simulink model "NDI"  (R2022a)
settings: Solver=ode4  StartTime=0  StopTime=100  FixedStep=fcs.Ts  RelTol=1e-3
undefined symbols (not defined in the file or in its folder): Aactuator, ac, AeroCoeff, ControlAllocation, DUmax, DUmin, EngineTable, F, fcs, ft, g, hground, IC, kg, LandingGear, Light, m, MIL, Mode_deflection_aileron, Mode_deflection_elevator, Mode_deflection_rudder, Mode_deflection_TVC_y, Mode_deflection_TVC_z, N, Ninv_2nozzle, Ninv_no_nozzle, PIController, s, Sensor, sigbuilder_block, slug, state0, sysID_DAQ, sysID_OBES, Umax_2nozzle, Umax_no_nozzle, Umin_2nozzle, Umin_no_nozzle, WMM2020
libraries: aerolibconvert2 x31, slpidlib x11, simulink x6, sharedutil x4, aerolibatmos2 x3, aerolibwind2 x3, aerolibbdyn x3, aerolibgravity2 x2, sharedtransform x1
(part 5 of 13)

== system NDI/F-16 Vehicle Systems Model/pqr NDI Controller ==
  note: $\hat{L}, \hat{M}, \hat{N}$
  note: 【有向量噴嘴控制】
      | (註：有/無向量噴嘴的差異之處在於 "粉紅色模塊" 的內容)
  note: 1  gp_dra1
      |     gp_dla1
      |     gp_dre1
      |     gp_dle1
      |     gp_dr1
      |     gp_dra2
      |     gp_dla2
      |     gp_dre2
      |     gp_dle2
      |     gp_dr2
      |
      | 11 gq_dra
      |      gq_dla
      |      gq_dre
      |      gq_dle
      |
      | 15 gr_dra1
      |      gr_dla1
      |      gr_dre1
      |      gr_dle1
      |      gr_dr1
      |      gr_dra2
      |      gr_dla2
      |      gr_dre2
      |      gr_dle2
      |      gr_dr2
  note: $g_1 {\left({\overset{-}{x} }_1 \right)}={\left[\begin{array}{ccccccccc} g_{p_{\delta_{ra} } } & g_{p_{\delta_{la} } } & g_{p_{\delta_{re} } } & g_{p_{\delta_{le} } } & g_{p_{\delta_r } } & g_{p_{\delta_{ry} } } & g_{p_{\delta_{rz} } } & g_{p_{\delta_{ly} } } & g_{p_{\delta_{lz} } } \\ g_{q_{\delta_{ra} } } & g_{q_{\delta_{la} } } & g_{q_{\delta_{re} } } & g_{q_{\delta_{le} } } & 0 & g_{q_{\delta_{ry} } } & 0 & g_{q_{\delta_{ly} } } & 0 \\ g_{r_{\delta_{ra} } } & g_{r_{\delta_{la} } } & g_{r_{\delta_{re} } } & g_{r_{\delta_{le} } } & g_{r_{\delta_r } } & g_{r_{\delta_{ry} } } & g_{r_{\delta_{rz} } } & g_{r_{\delta_{ly} } } & g_{r_{\delta_{lz} } } \end{array}\right]}$
  note: 選擇偏轉模式
  coef M : Inport
  control g : Inport  Port=2
  pqr dot desire : Inport  Port=3
  p q r : Inport  Port=4
  In Bus Element : Inport  Port=5  PortName=PlantData  Element=PropBus.T
  In Bus Element12 : Inport  Port=5  PortName=PlantData  Element=alpha
  In Bus Element3 : Inport  Port=5  PortName=PlantData  Element=Vt
  In Bus Element14 : Inport  Port=5  PortName=PlantData  Element=altitude
  " f1" : MATLAB Function  TreatAsAtomicUnit=on
  Angle Conversion : aerolibconvert2/Angle Conversion  IU=rad  OU=deg
  Constant : Constant  Value=0
  Constant1 : Constant  Value=N
  Control Allocation : Subsystem
  Demux : Demux  Outputs=9
  Ix(slug*ft^2)1 : Constant  Value=ac.Ix
  Ixz(slug*ft^2)1 : Constant  Value=ac.Ixz
  Iy(slug*ft^2)1 : Constant  Value=ac.Iy
  Iz(slug*ft^2)1 : Constant  Value=ac.Iz
  MakeINMAT : Subsystem
  Mode_deflection : Subsystem
  Sum : Sum  Inputs=+-|
  To Workspace3 : ToWorkspace  VariableName=upast  SaveFormat=Timeseries  SampleTime=-1
  Unit Delay : UnitDelay  InitialCondition=[0 0 0 0 0 0 0 0 0]  SampleTime=fcs.Ts  HasFrameUpgradeWarning=on
  control matrix g1 : Subsystem
  left_rudder : Terminator
  "TVC_ry " : Outport  VectorParamsAs1DForOutWhenUnconnected=off
  TVC_rz : Outport  Port=2  VectorParamsAs1DForOutWhenUnconnected=off
  "TVC_ly " : Outport  Port=3  VectorParamsAs1DForOutWhenUnconnected=off
  "TVC_lz " : Outport  Port=4  VectorParamsAs1DForOutWhenUnconnected=off
  right_aileron : Outport  Port=5  VectorParamsAs1DForOutWhenUnconnected=off
  left_aileron : Outport  Port=6  VectorParamsAs1DForOutWhenUnconnected=off
  right_elevator : Outport  Port=7  VectorParamsAs1DForOutWhenUnconnected=off
  left_elevator : Outport  Port=8  VectorParamsAs1DForOutWhenUnconnected=off
  rudder : Outport  Port=9  VectorParamsAs1DForOutWhenUnconnected=off
  wires:
  coef M/1 -> " f1"/1(moments)
  p q r/1 -> " f1"/2(pqr)
  " f1"/1(f1) -> Sum/2
  pqr dot desire/1 -> Sum/1
  In Bus Element/1 -> control matrix g1/2(Thrust T)
  control g/1 -> control matrix g1/1(coef g)
  Iy(slug*ft^2)1/1 -> " f1"/4(Iy)
  Ix(slug*ft^2)1/1 -> " f1"/3(Ix)
  Iz(slug*ft^2)1/1 -> " f1"/5(Iz)
  Ixz(slug*ft^2)1/1 -> " f1"/6(Ixz)
  MakeINMAT/1(IN_MAT) -> Control Allocation/1(IN_MAT1)
  Sum/1 -> Control Allocation/5(y_bar), MakeINMAT/1(f1)
  control matrix g1/1(g1) -> Control Allocation/6(g1), MakeINMAT/2(g1)
  Control Allocation/1(Du) -> Unit Delay/1, To Workspace3/1, Demux/1
  Unit Delay/1 -> MakeINMAT/3(In3)
  In Bus Element3/1 -> Control Allocation/3(Vt (ft/s))
  In Bus Element14/1 -> Control Allocation/4(altitude (ft))
  Constant/1 -> Mode_deflection/6(dlr)
  Constant1/1 -> Control Allocation/7(N)
  Demux/9 -> Mode_deflection/10(dlz)
  Demux/1 -> Mode_deflection/1(dra)
  Demux/2 -> Mode_deflection/2(dla)
  Demux/5 -> Mode_deflection/5(drr)
  Demux/4 -> Mode_deflection/4(dle)
  Demux/8 -> Mode_deflection/9(dly)
  Demux/6 -> Mode_deflection/7(dry)
  Demux/3 -> Mode_deflection/3(dre)
  Demux/7 -> Mode_deflection/8(drz)
  Mode_deflection/9("TVC_ly ") -> "TVC_ly "/1
  Mode_deflection/10("TVC_lz ") -> "TVC_lz "/1
  Mode_deflection/7("TVC_ry ") -> "TVC_ry "/1
  Mode_deflection/8(TVC_rz) -> TVC_rz/1
  Mode_deflection/2(left_aileron) -> left_aileron/1
  Mode_deflection/4(left_elevator) -> left_elevator/1
  Mode_deflection/6(left_rudder) -> left_rudder/1
  Mode_deflection/1(right_aileron) -> right_aileron/1
  Mode_deflection/3(right_elevator) -> right_elevator/1
  Mode_deflection/5(rudder) -> rudder/1
  In Bus Element12/1 -> Angle Conversion/1
  Angle Conversion/1 -> Control Allocation/2(alpha (deg))

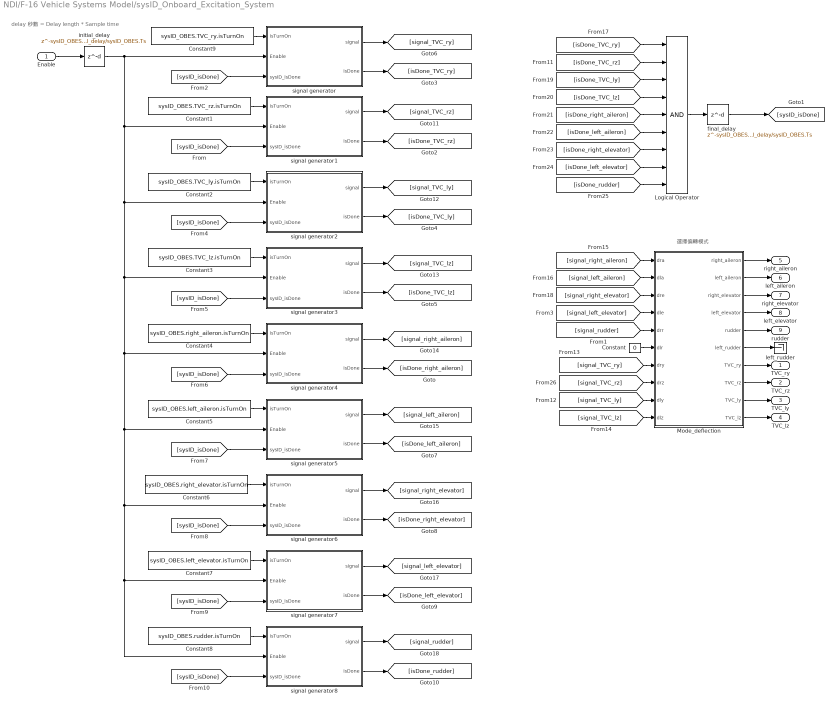
== system NDI/F-16 Vehicle Systems Model/sysID_Onboard_Excitation_System ==
  note: delay 秒數 = Delay length * Sample time
  note: 選擇偏轉模式
  Enable : Inport
  Constant : Constant  Value=0
  Constant1 : Constant  Value=sysID_OBES.TVC_rz.isTurnOn
  Constant2 : Constant  Value=sysID_OBES.TVC_ly.isTurnOn
  Constant3 : Constant  Value=sysID_OBES.TVC_lz.isTurnOn
  Constant4 : Constant  Value=sysID_OBES.right_aileron.isTurnOn
  Constant5 : Constant  Value=sysID_OBES.left_aileron.isTurnOn
  Constant6 : Constant  Value=sysID_OBES.right_elevator.isTurnOn
  Constant7 : Constant  Value=sysID_OBES.left_elevator.isTurnOn
  Constant8 : Constant  Value=sysID_OBES.rudder.isTurnOn
  Constant9 : Constant  Value=sysID_OBES.TVC_ry.isTurnOn
  Logical Operator : Logic  Inputs=9  AllPortsSameDT=off  OutDataTypeStr=boolean
  Mode_deflection : Subsystem
  final_delay : Delay  DelayLength=sysID_OBES.final_delay/sysID_OBES.Ts  SampleTime=sysID_OBES.Ts
  initial_delay : Delay  DelayLength=sysID_OBES.initial_delay/sysID_OBES.Ts  SampleTime=sysID_OBES.Ts
  left_rudder : Terminator
  signal generator : Subsystem  TreatAsAtomicUnit=on
  signal generator1 : Subsystem  TreatAsAtomicUnit=on
  signal generator2 : Subsystem  TreatAsAtomicUnit=on
  signal generator3 : Subsystem  TreatAsAtomicUnit=on
  signal generator4 : Subsystem  TreatAsAtomicUnit=on
  signal generator5 : Subsystem  TreatAsAtomicUnit=on
  signal generator6 : Subsystem  TreatAsAtomicUnit=on
  signal generator7 : Subsystem  TreatAsAtomicUnit=on
  signal generator8 : Subsystem  TreatAsAtomicUnit=on
  TVC_ry : Outport
  TVC_rz : Outport  Port=2
  TVC_ly : Outport  Port=3
  TVC_lz : Outport  Port=4
  right_aileron : Outport  Port=5
  left_aileron : Outport  Port=6
  right_elevator : Outport  Port=7
  left_elevator : Outport  Port=8
  rudder : Outport  Port=9
  wires:
  Logical Operator/1 -> final_delay/1
  final_delay/1 -> [sysID_isDone]
  signal generator1/2(isDone) -> [isDone_TVC_rz]
  [sysID_isDone] -> signal generator1/3(sysID_isDone)
  Enable/1 -> initial_delay/1
  signal generator/2(isDone) -> [isDone_TVC_ry]
  [sysID_isDone] -> signal generator/3(sysID_isDone)
  signal generator2/2(isDone) -> [isDone_TVC_ly]
  [sysID_isDone] -> signal generator2/3(sysID_isDone)
  signal generator3/2(isDone) -> [isDone_TVC_lz]
  [sysID_isDone] -> signal generator3/3(sysID_isDone)
  signal generator4/2(isDone) -> [isDone_right_aileron]
  [sysID_isDone] -> signal generator4/3(sysID_isDone)
  signal generator5/2(isDone) -> [isDone_left_aileron]
  [sysID_isDone] -> signal generator5/3(sysID_isDone)
  [sysID_isDone] -> signal generator6/3(sysID_isDone)
  signal generator6/2(isDone) -> [isDone_right_elevator]
  [sysID_isDone] -> signal generator7/3(sysID_isDone)
  signal generator7/2(isDone) -> [isDone_left_elevator]
  [sysID_isDone] -> signal generator8/3(sysID_isDone)
  initial_delay/1 -> signal generator1/2(Enable), signal generator2/2(Enable), signal generator3/2(Enable), signal generator4/2(Enable), signal generator5/2(Enable), signal generator6/2(Enable), signal generator8/2(Enable), signal generator7/2(Enable), signal generator/2(Enable)
  signal generator8/2(isDone) -> [isDone_rudder]
  Constant1/1 -> signal generator1/1(isTurnOn)
  Constant2/1 -> signal generator2/1(isTurnOn)
  Constant3/1 -> signal generator3/1(isTurnOn)
  Constant4/1 -> signal generator4/1(isTurnOn)
  Constant5/1 -> signal generator5/1(isTurnOn)
  Constant6/1 -> signal generator6/1(isTurnOn)
  Constant7/1 -> signal generator7/1(isTurnOn)
  Constant8/1 -> signal generator8/1(isTurnOn)
  Constant/1 -> Mode_deflection/6(dlr)
  Constant9/1 -> signal generator/1(isTurnOn)
  [isDone_TVC_ly] -> Logical Operator/3
  [isDone_TVC_lz] -> Logical Operator/4
  [isDone_right_aileron] -> Logical Operator/5
  [isDone_left_aileron] -> Logical Operator/6
  [isDone_right_elevator] -> Logical Operator/7
  [isDone_left_elevator] -> Logical Operator/8
  [signal_TVC_ry] -> Mode_deflection/7(dry)
  [isDone_rudder] -> Logical Operator/9
  [signal_TVC_ly] -> Mode_deflection/9(dly)
  [isDone_TVC_ry] -> Logical Operator/1
  [signal_TVC_lz] -> Mode_deflection/10(dlz)
  [signal_right_aileron] -> Mode_deflection/1(dra)
  [signal_left_aileron] -> Mode_deflection/2(dla)
  [signal_right_elevator] -> Mode_deflection/3(dre)
  [signal_left_elevator] -> Mode_deflection/4(dle)
  [signal_rudder] -> Mode_deflection/5(drr)
  [signal_TVC_rz] -> Mode_deflection/8(drz)
  [isDone_TVC_rz] -> Logical Operator/2
  Mode_deflection/9("TVC_ly ") -> TVC_ly/1
  Mode_deflection/10("TVC_lz ") -> TVC_lz/1
  Mode_deflection/7("TVC_ry ") -> TVC_ry/1
  Mode_deflection/8(TVC_rz) -> TVC_rz/1
  Mode_deflection/2(left_aileron) -> left_aileron/1
  Mode_deflection/4(left_elevator) -> left_elevator/1
  Mode_deflection/6(left_rudder) -> left_rudder/1
  Mode_deflection/1(right_aileron) -> right_aileron/1
  Mode_deflection/3(right_elevator) -> right_elevator/1
  Mode_deflection/5(rudder) -> rudder/1
  signal generator1/1(signal) -> [signal_TVC_rz]
  signal generator2/1(signal) -> [signal_TVC_ly]
  signal generator3/1(signal) -> [signal_TVC_lz]
  signal generator4/1(signal) -> [signal_right_aileron]
  signal generator5/1(signal) -> [signal_left_aileron]
  signal generator6/1(signal) -> [signal_right_elevator]
  signal generator7/1(signal) -> [signal_left_elevator]
  signal generator8/1(signal) -> [signal_rudder]
  signal generator/1(signal) -> [signal_TVC_ry]

== system NDI/F-16 Vehicle Systems Model/μαβ NDI Controller ==
  aero F : Inport
  μαβ dot desire : Inport  Port=2
  LGxyz : Inport  Port=3
  gravity : Inport  Port=4
  In Bus Element2 : Inport  Port=5  PortName=AirData  Element=alpha
  In Bus Element4 : Inport  Port=5  PortName=AirData  Element=alpha
  In Bus Element3 : Inport  Port=5  PortName=AirData  Element=beta
  In Bus Element5 : Inport  Port=5  PortName=AirData  Element=beta
  In Bus Element6 : Inport  Port=5  PortName=AirData  Element=mu
  In Bus Element7 : Inport  Port=5  PortName=AirData  Element=Vt
  In Bus Element8 : Inport  Port=5  PortName=AirData  Element=gamma
  In Bus Element : Inport  Port=6  PortName=PlantData  Element=PropBus.T
  In Bus Element1 : Inport  Port=6  PortName=PlantData  Element=chi
  Mux : Mux  Inputs=5
  Sum : Sum  Inputs=+-|
  attitude NDI : MATLAB Function  TreatAsAtomicUnit=on
  command matrix : Subsystem
  f2 : Subsystem
  pc : Outport  VectorParamsAs1DForOutWhenUnconnected=off
  qc : Outport  Port=2  VectorParamsAs1DForOutWhenUnconnected=off
  rc : Outport  Port=3  VectorParamsAs1DForOutWhenUnconnected=off
  D : Outport  Port=4  VectorParamsAs1DForOutWhenUnconnected=off
  Y : Outport  Port=5  VectorParamsAs1DForOutWhenUnconnected=off
  L : Outport  Port=6  VectorParamsAs1DForOutWhenUnconnected=off
  wires:
  f2/1(f2) -> Sum/2
  μαβ dot desire/1 -> Sum/1
  Sum/1 -> attitude NDI/1(y_bar)
  attitude NDI/1(p_c) -> pc/1
  attitude NDI/2(q_c) -> qc/1
  attitude NDI/3(r_c) -> rc/1
  command matrix/1(g2) -> attitude NDI/2(g2)
  Mux/1 -> f2/1(aero V)  "V, α, β, μ, γ"
  In Bus Element/1 -> f2/4(Thrust)
  aero F/1 -> f2/2(X,Y,Z)
  f2/2(D) -> D/1
  f2/3(Y) -> Y/1
  f2/4(L) -> L/1
  gravity/1 -> f2/3(gravity)
  In Bus Element2/1 -> command matrix/1(α)
  In Bus Element3/1 -> command matrix/2(β)
  In Bus Element5/1 -> Mux/3
  In Bus Element4/1 -> Mux/2
  In Bus Element6/1 -> Mux/4
  In Bus Element7/1 -> Mux/1
  In Bus Element8/1 -> Mux/5
  LGxyz/1 -> f2/5(LGxyz)
  In Bus Element1/1 -> f2/6(chi)

== system NDI/F-16 Vehicle Systems Model/庭宇 6.3節短場降落(模擬秒數設定:inf) ==
  Demux : Demux  Tag=STV Demux  Outputs=5
      settings: DisplayOption=none
  FromWs : FromWorkspace  Tag=STV FromWs  VariableName=tuvar
      SigBuilderData=|
      | common.afterFinalStr = 'Extrapolate'
      | common.sampleTime = 0
      | dataSet.timeRange = [0 120]
      | dataSet.name = 'Group 1'
      | sbobj.Groups.Name = 'Group 1'
      | sbobj.Groups.Signals(1).Name = 'Vt'
      | sbobj.Groups.Signals(1).XData = [0 5 6.2 7.35 8.3 9.05 10.05 11.2 13.1 14.75 15 16.85 18.75 19.63 20 22.2 23.5 25 26.65 30 31.65 40 50 60 67.4 80 94.8 107.7 120]
      | sbobj.Groups.Signals(1).YData = [287 287 286.6 286 285 284.6 283.9 283.4 281.8 279.8 279.4 277 274.8 273.8 273.3 270.3 269 268 266.5 264 263 258 252 248 246 220 197 110 0]
      | sbobj.Groups.Signals(2).Name = 'y_ft'
      | sbobj.Groups.Signals(2).XData = [0 120]
      | sbobj.Groups.Signals(2).YData = [0 0]
      | sbobj.Groups.Signals(3).Name = 'h_ft'
      | sbobj.Groups.Signals(3).XData = [0 60 80.12 94 100 120]
      | sbobj.Groups.Signals(3).YData = [1000 100 6.1418 6.1418 5.9161 5.9161]
      | sbobj.Groups.Signals(4).Name = 'SB_deg'
      | sbobj.Groups.Signals(4).XData = [0 100 100 120]
      | sbobj.Groups.Signals(4).YData = [40 40 60 60]
      | sbobj.Groups.Signals(5).Name = 'LandingGear_down'
      | sbobj.Groups.Signals(5).XData = [0 120]
      | sbobj.Groups.Signals(5).YData = [1 1]
      | sbobj.Groups.TimeRange = [0 120]
  Vt : Outport  Tag=STV Outport  VectorParamsAs1DForOutWhenUnconnected=off
  y_ft : Outport  Tag=STV Outport  Port=2  VectorParamsAs1DForOutWhenUnconnected=off
  h_ft : Outport  Tag=STV Outport  Port=3  VectorParamsAs1DForOutWhenUnconnected=off
  SB_deg : Outport  Tag=STV Outport  Port=4
  LandingGear_down : Outport  Tag=STV Outport  Port=5
  wires:
  FromWs/1 -> Demux/1
  Demux/1 -> Vt/1
  Demux/2 -> y_ft/1
  Demux/3 -> h_ft/1
  Demux/4 -> SB_deg/1
  Demux/5 -> LandingGear_down/1

== system NDI/F-16 Vehicle Systems Model/落葉飄完整版(碩論6.7)1 ==
  Demux : Demux  Tag=STV Demux  Outputs=6
      settings: DisplayOption=none
  FromWs : FromWorkspace  Tag=STV FromWs  VariableName=tuvar
      SigBuilderData=|
      | common.afterFinalStr = 'Extrapolate'
      | common.sampleTime = 0
      | dataSet.timeRange = [0 70]
      | dataSet.name = 'Group 5'
      | sbobj.Groups.Name = 'Group 5'
      | sbobj.Groups.Signals(1).Name = 'thrust'
      | sbobj.Groups.Signals(1).XData = [0 2 4 5 6 8 9 10 12 20 25 30 35 40 70]
      | sbobj.Groups.Signals(1).YData = [5100 5100 600 200 200 200 265 3500 3500 3500 6000 15200 15200 10000 10000]
      | sbobj.Groups.Signals(2).Name = 'mu'
      | sbobj.Groups.Signals(2).XData = [0 2 8 10 12 20 30 40 55 67 70]
      | sbobj.Groups.Signals(2).YData = [0 0 0 0 0 90 90 0 80 0 0]
      | sbobj.Groups.Signals(3).Name = 'alpha'
      | sbobj.Groups.Signals(3).XData = [0 1 2 3 10 35 37 60 70]
      | sbobj.Groups.Signals(3).YData = [7 30 31 60 70 70 10 20 20]
      | sbobj.Groups.Signals(4).Name = 'beta'
      | sbobj.Groups.Signals(4).XData = [0 8 70]
      | sbobj.Groups.Signals(4).YData = [0 0 0]
      | sbobj.Groups.Signals(5).Name = 'speed brake'
      | sbobj.Groups.Signals(5).XData = [0 70]
      | sbobj.Groups.Signals(5).YData = [0 0]
      | sbobj.Groups.Signals(6).Name = 'LandingGear_down'
      | sbobj.Groups.Signals(6).XData = [0 70]
      | sbobj.Groups.Signals(6).YData = [1 1]
      | sbobj.Groups.TimeRange = [0 70]
  thrust : Outport  Tag=STV Outport
  mu : Outport  Tag=STV Outport  Port=2  VectorParamsAs1DForOutWhenUnconnected=off
  alpha : Outport  Tag=STV Outport  Port=3  VectorParamsAs1DForOutWhenUnconnected=off
  beta : Outport  Tag=STV Outport  Port=4  VectorParamsAs1DForOutWhenUnconnected=off
  speed brake : Outport  Tag=STV Outport  Port=5
  LandingGear_down : Outport  Tag=STV Outport  Port=6
  wires:
  FromWs/1 -> Demux/1
  Demux/1 -> thrust/1
  Demux/2 -> mu/1
  Demux/3 -> alpha/1
  Demux/4 -> beta/1
  Demux/5 -> speed brake/1
  Demux/6 -> LandingGear_down/1

== system NDI/F-16 Vehicle Systems Model/Aerodynamic1/Creating    qbar // ps ==
  h (ft) : Inport
  Vt (ft/s) : Inport  Port=2
  Constant2 : Constant
  Constant3 : Constant  Value=390
  Constant6 : Constant  Value=4.14
  Math Function : Math  Operator=pow  SignedPower=on
  Math Function1 : Math  Operator=square  SignedPower=on
  Product : Product  Inputs=/*  InputSameDT=on  SaturateOnIntegerOverflow=on  OutDataTypeStr=Inherit: Same as first input
  Product5 : Product  Inputs=**  InputSameDT=on  SaturateOnIntegerOverflow=on  OutDataTypeStr=Inherit: Same as first input
  Product6 : Product  Inputs=**  InputSameDT=on  SaturateOnIntegerOverflow=on  OutDataTypeStr=Inherit: Same as first input
  Sum3 : Sum  Inputs=+-|  InputSameDT=on  SaturateOnIntegerOverflow=on  OutDataTypeStr=Inherit: Same as first input
  Switch : Switch  Threshold=35000
  r2d2 : Gain  Gain=0.703e-5  SaturateOnIntegerOverflow=on  OutDataTypeStr=Inherit: Same as input  ParamDataTypeStr=Inherit: Same as input
  r2d3 : Gain  Gain=519  SaturateOnIntegerOverflow=on  OutDataTypeStr=Inherit: Same as input  ParamDataTypeStr=Inherit: Same as input
  r2d4 : Gain  Gain=0.5  SaturateOnIntegerOverflow=on  OutDataTypeStr=Inherit: Same as input  ParamDataTypeStr=Inherit: Same as input
  r2d5 : Gain  Gain=1715  SaturateOnIntegerOverflow=on  OutDataTypeStr=Inherit: Same as input  ParamDataTypeStr=Inherit: Same as input
  rho0 : Gain  Gain=2.377e-3  SaturateOnIntegerOverflow=on  OutDataTypeStr=Inherit: Same as input  ParamDataTypeStr=Inherit: Same as input
  qbar / ps : Outport  VectorParamsAs1DForOutWhenUnconnected=off
  wires:
  h (ft)/1 -> r2d2/1, Switch/2
  Sum3/1 -> Math Function/1, r2d3/1  "tfac"
  Constant3/1 -> Switch/1
  r2d3/1 -> Switch/3
  Constant6/1 -> Math Function/2
  rho0/1 -> Product5/1, Product6/2  "rho"
  r2d2/1 -> Sum3/2
  Constant2/1 -> Sum3/1
  Math Function/1 -> rho0/1
  Math Function1/1 -> Product5/2
  Switch/1 -> r2d5/1  "temp"
  r2d5/1 -> Product6/1
  Product6/1 -> Product/1  "ps"
  Product5/1 -> r2d4/1  "qbar"
  Product/1 -> qbar / ps/1
  Vt (ft/s)/1 -> Math Function1/1  "Vt (ft/s)"
  r2d4/1 -> Product/2

== system NDI/F-16 Vehicle Systems Model/Aerodynamic1/ISP  ==
  note: 1 T
      | 2 a (Speed of sound)
      | 3 P
      | 4 rho
      | 5 g
      | 6 mu (Coefficient of viscosity)
  h (ft) : Inport
  Vt (ft/s) : Inport  Port=2
  Demux : Demux  Outputs=[1,1,1,1,1,1]
      settings: DisplayOption=none
  Divide1 : Product  Inputs=*/
  Length Conversion : aerolibconvert2/Length Conversion  IU=ft  OU=m
  MATLAB Function : MATLAB Function  TreatAsAtomicUnit=on
  Product : Product
  Square : Math  Operator=square  SignedPower=on
  r2d1 : Gain  Gain=0.5  SaturateOnIntegerOverflow=on  OutDataTypeStr=Inherit: Same as input  ParamDataTypeStr=Inherit: Same as input
  r2d3 : Gain  Gain=3.2808399  SaturateOnIntegerOverflow=on  OutDataTypeStr=Inherit: Same as input  ParamDataTypeStr=Inherit: Same as input
  r2d4 : Gain  Gain=0.00194032033  SaturateOnIntegerOverflow=on  OutDataTypeStr=Inherit: Same as input  ParamDataTypeStr=Inherit: Same as input
  T(K) : Outport  VectorParamsAs1DForOutWhenUnconnected=off
  "Mach " : Outport  Port=2  VectorParamsAs1DForOutWhenUnconnected=off
  P(HPa) : Outport  Port=3  VectorParamsAs1DForOutWhenUnconnected=off
  "qbar " : Outport  Port=4  VectorParamsAs1DForOutWhenUnconnected=off
  rho : Outport  Port=5  VectorParamsAs1DForOutWhenUnconnected=off
  g (m/s^2) : Outport  Port=6  VectorParamsAs1DForOutWhenUnconnected=off
  mu : Outport  Port=7  VectorParamsAs1DForOutWhenUnconnected=off
  wires:
  r2d3/1 -> Divide1/2
  r2d1/1 -> Product/2
  Demux/4 -> rho/1, r2d4/1  "rho(kg/m^3)"
  Demux/2 -> r2d3/1  "a(m/s)"
  Demux/1 -> T(K)/1  "T(K)"
  r2d4/1 -> r2d1/1
  Divide1/1 -> "Mach "/1
  Demux/5 -> g (m/s^2)/1  "g (m/s^2)"
  Demux/6 -> mu/1  "mu"
  Product/1 -> "qbar "/1
  Square/1 -> Product/1
  Vt (ft/s)/1 -> Square/1, Divide1/1
  Demux/3 -> P(HPa)/1  "P(Pa)"
  h (ft)/1 -> Length Conversion/1
  Length Conversion/1 -> MATLAB Function/1(h)
  MATLAB Function/1(ISP_output) -> Demux/1

== system NDI/F-16 Vehicle Systems Model/Aerodynamic1/NDI Aerofynamic Coefficients ==
  note: leading-edge flaps
      | 前緣襟翼
  note: speed brake
      | 減速板
  note: Total Velocity
  note: 未建模，缺少數據
  note: ${\left(1-\frac{\delta_{LEF} }{25°}\right)}$
  alpha (deg) : Inport
  beta (deg) : Inport  Port=2
  LEF (deg) : Inport  Port=3
  right elevator (deg) : Inport  Port=4
  left elevator (deg) : Inport  Port=5
  right alieron (deg) : Inport  Port=6
  left alieron (deg) : Inport  Port=7
  rudder (deg) : Inport  Port=8
  SB (deg) : Inport  Port=9  Unit=deg
  Vt (ft/s) : Inport  Port=10
  p (rad/s) : Inport  Port=11
  q (rad/s) : Inport  Port=12
  r (rad/s) : Inport  Port=13
  GearAngle : Inport  Port=14
  h_AGL : Inport  Port=15
  Add : Sum  Inputs=-+
  CXT : Subsystem
  CYT : Subsystem
  CZT : Subsystem
  ClT : Subsystem
  CmT : Subsystem
  CnT : Subsystem
  Constant3 : Constant
  Divide2 : Product  Inputs=**/
  Divide3 : Product  Inputs=**/
  Divide4 : Product  Inputs=**/
  Gain1 : Gain  Gain=2
  Ground Effects : Subsystem  Commented=on
  Landing Gear Effects : Subsystem  Commented=on
  Mux : Mux  Inputs=2
  Mux1 : Mux  Inputs=2
  Terminator : Terminator  Commented=on
  Terminator1 : Terminator  Commented=on
  b(ft) : Constant  Value=ac.b
  cbar(ft) : Constant  Value=ac.cbar
  center of gravity as a fraction of cbar : Constant  Value=ac.x_cg
  r2d1 : Gain  Gain=1/25  SaturateOnIntegerOverflow=on  OutDataTypeStr=Inherit: Same as input  ParamDataTypeStr=Inherit: Same as input
  r2d2 : Gain  Gain=1/60  SaturateOnIntegerOverflow=on  OutDataTypeStr=Inherit: Same as input  ParamDataTypeStr=Inherit: Same as input
  r2d3 : Gain  Gain=1/20  SaturateOnIntegerOverflow=on  OutDataTypeStr=Inherit: Same as input  ParamDataTypeStr=Inherit: Same as input
  r2d4 : Gain  Gain=1/30  SaturateOnIntegerOverflow=on  OutDataTypeStr=Inherit: Same as input  ParamDataTypeStr=Inherit: Same as input
  r2d5 : Gain  Gain=1/20  SaturateOnIntegerOverflow=on  OutDataTypeStr=Inherit: Same as input  ParamDataTypeStr=Inherit: Same as input
  reference center of gravity as a fraction of cbar : Constant  Value=ac.x_cg_ref
  CX_T : Outport  VectorParamsAs1DForOutWhenUnconnected=off
  CY_T : Outport  Port=2  VectorParamsAs1DForOutWhenUnconnected=off
  CZ_T : Outport  Port=3  VectorParamsAs1DForOutWhenUnconnected=off
  Cl_T_hat : Outport  Port=4  VectorParamsAs1DForOutWhenUnconnected=off
  Cm_T_hat : Outport  Port=5  VectorParamsAs1DForOutWhenUnconnected=off
  Cn_T_hat : Outport  Port=6  VectorParamsAs1DForOutWhenUnconnected=off
  gp : Outport  Port=7  VectorParamsAs1DForOutWhenUnconnected=off
  gq : Outport  Port=8  VectorParamsAs1DForOutWhenUnconnected=off
  gr : Outport  Port=9  VectorParamsAs1DForOutWhenUnconnected=off
  wires:
  alpha (deg)/1 -> CXT/1(alpha (deg)), CnT/1(alpha (deg)), CmT/1(alpha (deg)), ClT/1(alpha (deg)), CZT/1(alpha (deg)), CYT/1(alpha (deg))
  beta (deg)/1 -> CXT/2(beta (deg)), CnT/2(beta (deg)), CmT/2(beta (deg)), ClT/2(beta (deg)), CZT/2(beta (deg)), CYT/2(beta (deg))
  right elevator (deg)/1 -> CXT/3(right elevator (deg)), CnT/3(right elevator (deg)), CmT/3(right elevator (deg)), ClT/3(right elevator (deg)), CZT/3(right elevator (deg))
  Vt (ft/s)/1 -> Gain1/1
  p (rad/s)/1 -> Divide4/1  "p"
  q (rad/s)/1 -> Divide2/1  "q"
  r (rad/s)/1 -> Divide3/1  "r"
  b(ft)/1 -> Divide4/2, Divide3/2, CnT/11(b)  "b"
  cbar(ft)/1 -> Divide2/2, CnT/10(cbar)  "cbar"
  Add/1 -> CXT/5(dlef), CnT/5(dlef), CmT/5(dlef), ClT/5(dlef), CZT/5(dlef), CYT/3(dlef)  "dlef"
  left alieron (deg)/1 -> r2d3/1
  rudder (deg)/1 -> r2d4/1
  Divide2/1 -> CXT/6(qc_2v), CZT/6(qc_2v), CmT/6(qc_2v)  "qc_2v"
  r2d4/1 -> CYT/6(drud)
  Divide3/1 -> CnT/6(rb_2v), CYT/7(rb_2v), ClT/6(rb_2v)  "rb_2v"
  Divide4/1 -> CnT/7(pb_2v), CYT/8(pb_2v), ClT/7(pb_2v)  "pb_2v"
  reference center of gravity as a fraction of cbar/1 -> CmT/7(x_cg_ref), CnT/8(x_cg_ref)
  center of gravity as a fraction of cbar/1 -> CmT/8(x_cg), CnT/9(x_cg)
  CZT/1(Cz_tot_plus) -> CmT/10(Cz_tot_plus)
  CZT/2(Cz_tot_minus) -> CmT/11(Cz_tot_minus)
  CYT/2(Cy_tot_n_mom) -> CnT/12(Cy_tot_n_mom)
  CYT/3(Cy_tot_n_da) -> CnT/13(Cy_tot_n_da)
  CYT/4(Cy_tot_n_dr) -> CnT/14(Cy_tot_n_dr)
  SB (deg)/1 -> r2d2/1
  CXT/1(Cx_tot) -> CX_T/1
  CYT/1(Cy_tot) -> CY_T/1
  CZT/5(Cz_tot) -> CZ_T/1
  CnT/1(Cn_tot_hat) -> Cn_T_hat/1
  CmT/1(Cm_tot_hat) -> Cm_T_hat/1
  ClT/1(Cl_tot_hat) -> Cl_T_hat/1
  LEF (deg)/1 -> r2d1/1
  r2d2/1 -> CXT/7(sb), CmT/12(sb), CZT/7(sb)
  Gain1/1 -> Divide3/3, Divide2/3, Divide4/3  "2v"
  Landing Gear Effects/1(Coeff) -> Terminator/1
  h_AGL/1 -> Ground Effects/3(h_AGL)
  Ground Effects/1(Coeff) -> Terminator1/1
  GearAngle/1 -> Landing Gear Effects/3(Landing Gear Angle)
  right alieron (deg)/1 -> r2d5/1
  r2d5/1 -> CXT/8(right aileron), CYT/4(right aileron)
  r2d3/1 -> CYT/5(left aileron), CXT/9(left aileron)
  r2d1/1 -> Add/1
  Constant3/1 -> Add/2
  left elevator (deg)/1 -> CXT/4(left elevator (deg)), CnT/4(left elevator (deg)), CmT/4(left elevator (deg)), ClT/4(left elevator (deg)), CZT/4(left elevator (deg))
  Mux1/1 -> gr/1
  CmT/3(gq) -> gq/1
  CnT/3(gr2) -> Mux1/2
  ClT/3(gr1) -> Mux1/1
  CnT/2(gp2) -> Mux/2
  Mux/1 -> gp/1
  ClT/2(gp1) -> Mux/1
  CZT/6(Cz_tot_hat) -> CmT/9(Cz_tot_hat)
  CYT/5(Cy_tot_n_de) -> CnT/15(Cy_tot_n_de)
  CZT/3(Cz_tot_m_de) -> CmT/13(Cz_tot_m_de)
  CZT/4(Cz_tot_m_da) -> CmT/14(Cz_tot_m_da)

== system NDI/F-16 Vehicle Systems Model/Aerodynamic2/Creating    qbar // ps ==
  h (ft) : Inport
  Vt (ft/s) : Inport  Port=2
  Constant2 : Constant
  Constant3 : Constant  Value=390
  Constant6 : Constant  Value=4.14
  Math Function : Math  Operator=pow  SignedPower=on
  Math Function1 : Math  Operator=square  SignedPower=on
  Product : Product  Inputs=/*  InputSameDT=on  SaturateOnIntegerOverflow=on  OutDataTypeStr=Inherit: Same as first input
  Product5 : Product  Inputs=**  InputSameDT=on  SaturateOnIntegerOverflow=on  OutDataTypeStr=Inherit: Same as first input
  Product6 : Product  Inputs=**  InputSameDT=on  SaturateOnIntegerOverflow=on  OutDataTypeStr=Inherit: Same as first input
  Sum3 : Sum  Inputs=+-|  InputSameDT=on  SaturateOnIntegerOverflow=on  OutDataTypeStr=Inherit: Same as first input
  Switch : Switch  Threshold=35000
  r2d2 : Gain  Gain=0.703e-5  SaturateOnIntegerOverflow=on  OutDataTypeStr=Inherit: Same as input  ParamDataTypeStr=Inherit: Same as input
  r2d3 : Gain  Gain=519  SaturateOnIntegerOverflow=on  OutDataTypeStr=Inherit: Same as input  ParamDataTypeStr=Inherit: Same as input
  r2d4 : Gain  Gain=0.5  SaturateOnIntegerOverflow=on  OutDataTypeStr=Inherit: Same as input  ParamDataTypeStr=Inherit: Same as input
  r2d5 : Gain  Gain=1715  SaturateOnIntegerOverflow=on  OutDataTypeStr=Inherit: Same as input  ParamDataTypeStr=Inherit: Same as input
  rho0 : Gain  Gain=2.377e-3  SaturateOnIntegerOverflow=on  OutDataTypeStr=Inherit: Same as input  ParamDataTypeStr=Inherit: Same as input
  qbar / ps : Outport  VectorParamsAs1DForOutWhenUnconnected=off
  wires:
  h (ft)/1 -> r2d2/1, Switch/2
  Sum3/1 -> Math Function/1, r2d3/1  "tfac"
  Constant3/1 -> Switch/1
  r2d3/1 -> Switch/3
  Constant6/1 -> Math Function/2
  rho0/1 -> Product5/1, Product6/2  "rho"
  r2d2/1 -> Sum3/2
  Constant2/1 -> Sum3/1
  Math Function/1 -> rho0/1
  Math Function1/1 -> Product5/2
  Switch/1 -> r2d5/1  "temp"
  r2d5/1 -> Product6/1
  Product6/1 -> Product/1  "ps"
  Product5/1 -> r2d4/1  "qbar"
  Product/1 -> qbar / ps/1
  Vt (ft/s)/1 -> Math Function1/1  "Vt (ft/s)"
  r2d4/1 -> Product/2

== system NDI/F-16 Vehicle Systems Model/Aerodynamic2/ISP  ==
  note: 1 T
      | 2 a (Speed of sound)
      | 3 P
      | 4 rho
      | 5 g
      | 6 mu (Coefficient of viscosity)
  h (ft) : Inport
  Vt (ft/s) : Inport  Port=2
  Demux : Demux  Outputs=[1,1,1,1,1,1]
      settings: DisplayOption=none
  Divide1 : Product  Inputs=*/
  Length Conversion : aerolibconvert2/Length Conversion  IU=ft  OU=m
  MATLAB Function : MATLAB Function  TreatAsAtomicUnit=on
  Product : Product
  Square : Math  Operator=square  SignedPower=on
  r2d1 : Gain  Gain=0.5  SaturateOnIntegerOverflow=on  OutDataTypeStr=Inherit: Same as input  ParamDataTypeStr=Inherit: Same as input
  r2d3 : Gain  Gain=3.2808399  SaturateOnIntegerOverflow=on  OutDataTypeStr=Inherit: Same as input  ParamDataTypeStr=Inherit: Same as input
  r2d4 : Gain  Gain=0.00194032033  SaturateOnIntegerOverflow=on  OutDataTypeStr=Inherit: Same as input  ParamDataTypeStr=Inherit: Same as input
  T(K) : Outport  VectorParamsAs1DForOutWhenUnconnected=off
  "Mach " : Outport  Port=2  VectorParamsAs1DForOutWhenUnconnected=off
  P(HPa) : Outport  Port=3  VectorParamsAs1DForOutWhenUnconnected=off
  "qbar " : Outport  Port=4  VectorParamsAs1DForOutWhenUnconnected=off
  rho : Outport  Port=5  VectorParamsAs1DForOutWhenUnconnected=off
  g (m/s^2) : Outport  Port=6  VectorParamsAs1DForOutWhenUnconnected=off
  mu : Outport  Port=7  VectorParamsAs1DForOutWhenUnconnected=off
  wires:
  r2d3/1 -> Divide1/2
  r2d1/1 -> Product/2
  Demux/4 -> rho/1, r2d4/1  "rho(kg/m^3)"
  Demux/2 -> r2d3/1  "a(m/s)"
  Demux/1 -> T(K)/1  "T(K)"
  r2d4/1 -> r2d1/1
  Divide1/1 -> "Mach "/1
  Demux/5 -> g (m/s^2)/1  "g (m/s^2)"
  Demux/6 -> mu/1  "mu"
  Product/1 -> "qbar "/1
  Square/1 -> Product/1
  Vt (ft/s)/1 -> Square/1, Divide1/1
  Demux/3 -> P(HPa)/1  "P(Pa)"
  h (ft)/1 -> Length Conversion/1
  Length Conversion/1 -> MATLAB Function/1(h)
  MATLAB Function/1(ISP_output) -> Demux/1

== system NDI/F-16 Vehicle Systems Model/Aerodynamic2/NDI Aerofynamic Coefficients ==
  note: leading-edge flaps
      | 前緣襟翼
  note: speed brake
      | 減速板
  note: Total Velocity
  note: 未建模，缺少數據
  note: ${\left(1-\frac{\delta_{LEF} }{25°}\right)}$
  alpha (deg) : Inport
  beta (deg) : Inport  Port=2
  LEF (deg) : Inport  Port=3
  right elevator (deg) : Inport  Port=4
  left elevator (deg) : Inport  Port=5
  right alieron (deg) : Inport  Port=6
  left alieron (deg) : Inport  Port=7
  rudder (deg) : Inport  Port=8
  SB (deg) : Inport  Port=9  Unit=deg
  Vt (ft/s) : Inport  Port=10
  p (rad/s) : Inport  Port=11
  q (rad/s) : Inport  Port=12
  r (rad/s) : Inport  Port=13
  GearAngle : Inport  Port=14
  h_AGL : Inport  Port=15
  Add : Sum  Inputs=-+
  CXT : Subsystem
  CYT : Subsystem
  CZT : Subsystem
  ClT : Subsystem
  CmT : Subsystem
  CnT : Subsystem
  Constant3 : Constant
  Divide2 : Product  Inputs=**/
  Divide3 : Product  Inputs=**/
  Divide4 : Product  Inputs=**/
  Gain1 : Gain  Gain=2
  Ground Effects : Subsystem  Commented=on
  Landing Gear Effects : Subsystem  Commented=on
  Mux : Mux  Inputs=2
  Mux1 : Mux  Inputs=2
  Terminator : Terminator  Commented=on
  Terminator1 : Terminator  Commented=on
  b(ft) : Constant  Value=ac.b
  cbar(ft) : Constant  Value=ac.cbar
  center of gravity as a fraction of cbar : Constant  Value=ac.x_cg
  r2d1 : Gain  Gain=1/25  SaturateOnIntegerOverflow=on  OutDataTypeStr=Inherit: Same as input  ParamDataTypeStr=Inherit: Same as input
  r2d2 : Gain  Gain=1/60  SaturateOnIntegerOverflow=on  OutDataTypeStr=Inherit: Same as input  ParamDataTypeStr=Inherit: Same as input
  r2d3 : Gain  Gain=1/20  SaturateOnIntegerOverflow=on  OutDataTypeStr=Inherit: Same as input  ParamDataTypeStr=Inherit: Same as input
  r2d4 : Gain  Gain=1/30  SaturateOnIntegerOverflow=on  OutDataTypeStr=Inherit: Same as input  ParamDataTypeStr=Inherit: Same as input
  r2d5 : Gain  Gain=1/20  SaturateOnIntegerOverflow=on  OutDataTypeStr=Inherit: Same as input  ParamDataTypeStr=Inherit: Same as input
  reference center of gravity as a fraction of cbar : Constant  Value=ac.x_cg_ref
  CX_T : Outport  VectorParamsAs1DForOutWhenUnconnected=off
  CY_T : Outport  Port=2  VectorParamsAs1DForOutWhenUnconnected=off
  CZ_T : Outport  Port=3  VectorParamsAs1DForOutWhenUnconnected=off
  Cl_T_hat : Outport  Port=4  VectorParamsAs1DForOutWhenUnconnected=off
  Cm_T_hat : Outport  Port=5  VectorParamsAs1DForOutWhenUnconnected=off
  Cn_T_hat : Outport  Port=6  VectorParamsAs1DForOutWhenUnconnected=off
  gp : Outport  Port=7  VectorParamsAs1DForOutWhenUnconnected=off
  gq : Outport  Port=8  VectorParamsAs1DForOutWhenUnconnected=off
  gr : Outport  Port=9  VectorParamsAs1DForOutWhenUnconnected=off
  wires:
  alpha (deg)/1 -> CXT/1(alpha (deg)), CnT/1(alpha (deg)), CmT/1(alpha (deg)), ClT/1(alpha (deg)), CZT/1(alpha (deg)), CYT/1(alpha (deg))
  beta (deg)/1 -> CXT/2(beta (deg)), CnT/2(beta (deg)), CmT/2(beta (deg)), ClT/2(beta (deg)), CZT/2(beta (deg)), CYT/2(beta (deg))
  right elevator (deg)/1 -> CXT/3(right elevator (deg)), CnT/3(right elevator (deg)), CmT/3(right elevator (deg)), ClT/3(right elevator (deg)), CZT/3(right elevator (deg))
  Vt (ft/s)/1 -> Gain1/1
  p (rad/s)/1 -> Divide4/1  "p"
  q (rad/s)/1 -> Divide2/1  "q"
  r (rad/s)/1 -> Divide3/1  "r"
  b(ft)/1 -> Divide4/2, Divide3/2, CnT/11(b)  "b"
  cbar(ft)/1 -> Divide2/2, CnT/10(cbar)  "cbar"
  Add/1 -> CXT/5(dlef), CnT/5(dlef), CmT/5(dlef), ClT/5(dlef), CZT/5(dlef), CYT/3(dlef)  "dlef"
  left alieron (deg)/1 -> r2d3/1
  rudder (deg)/1 -> r2d4/1
  Divide2/1 -> CXT/6(qc_2v), CZT/6(qc_2v), CmT/6(qc_2v)  "qc_2v"
  r2d4/1 -> CYT/6(drud)
  Divide3/1 -> CnT/6(rb_2v), CYT/7(rb_2v), ClT/6(rb_2v)  "rb_2v"
  Divide4/1 -> CnT/7(pb_2v), CYT/8(pb_2v), ClT/7(pb_2v)  "pb_2v"
  reference center of gravity as a fraction of cbar/1 -> CmT/7(x_cg_ref), CnT/8(x_cg_ref)
  center of gravity as a fraction of cbar/1 -> CmT/8(x_cg), CnT/9(x_cg)
  CZT/1(Cz_tot_plus) -> CmT/10(Cz_tot_plus)
  CZT/2(Cz_tot_minus) -> CmT/11(Cz_tot_minus)
  CYT/2(Cy_tot_n_mom) -> CnT/12(Cy_tot_n_mom)
  CYT/3(Cy_tot_n_da) -> CnT/13(Cy_tot_n_da)
  CYT/4(Cy_tot_n_dr) -> CnT/14(Cy_tot_n_dr)
  SB (deg)/1 -> r2d2/1
  CXT/1(Cx_tot) -> CX_T/1
  CYT/1(Cy_tot) -> CY_T/1
  CZT/5(Cz_tot) -> CZ_T/1
  CnT/1(Cn_tot_hat) -> Cn_T_hat/1
  CmT/1(Cm_tot_hat) -> Cm_T_hat/1
  ClT/1(Cl_tot_hat) -> Cl_T_hat/1
  LEF (deg)/1 -> r2d1/1
  r2d2/1 -> CXT/7(sb), CmT/12(sb), CZT/7(sb)
  Gain1/1 -> Divide3/3, Divide2/3, Divide4/3  "2v"
  Landing Gear Effects/1(Coeff) -> Terminator/1
  h_AGL/1 -> Ground Effects/3(h_AGL)
  Ground Effects/1(Coeff) -> Terminator1/1
  GearAngle/1 -> Landing Gear Effects/3(Landing Gear Angle)
  right alieron (deg)/1 -> r2d5/1
  r2d5/1 -> CXT/8(right aileron), CYT/4(right aileron)
  r2d3/1 -> CYT/5(left aileron), CXT/9(left aileron)
  r2d1/1 -> Add/1
  Constant3/1 -> Add/2
  left elevator (deg)/1 -> CXT/4(left elevator (deg)), CnT/4(left elevator (deg)), CmT/4(left elevator (deg)), ClT/4(left elevator (deg)), CZT/4(left elevator (deg))
  Mux1/1 -> gr/1
  CmT/3(gq) -> gq/1
  CnT/3(gr2) -> Mux1/2
  ClT/3(gr1) -> Mux1/1
  CnT/2(gp2) -> Mux/2
  Mux/1 -> gp/1
  ClT/2(gp1) -> Mux/1
  CZT/6(Cz_tot_hat) -> CmT/9(Cz_tot_hat)
  CYT/5(Cy_tot_n_de) -> CnT/15(Cy_tot_n_de)
  CZT/3(Cz_tot_m_de) -> CmT/13(Cz_tot_m_de)
  CZT/4(Cz_tot_m_da) -> CmT/14(Cz_tot_m_da)

== system NDI/F-16 Vehicle Systems Model/Landing_Control/Stateflow/Stop_Sliding.Stop_Simulation ==
  f : TriggerPort  TriggerType=function-call  VariantControl=(inherit)
      settings: CopyFcn=Stateflow.SLINSF.SimulinkMan.removeBlockPreDeleteFcn  PreDeleteFcn=Stateflow.SLINSF.SimulinkMan.unsafePredeleteFcn
  Constant : Constant
  Stop Simulation : Stop
  wires:
  Constant/1 -> Stop Simulation/1

== system NDI/F-16 Vehicle Systems Model/Pilot commands storehouse/J trun(deg) ==
  Demux : Demux  Tag=STV Demux  Outputs=5
      settings: DisplayOption=none
  FromWs : FromWorkspace  Tag=STV FromWs  VariableName=tuvar
      SigBuilderData=|
      | common.afterFinalStr = 'Extrapolate'
      | common.sampleTime = 0
      | dataSet.timeRange = [0 20]
      | dataSet.name = 'Group 5'
      | sbobj.Groups.Name = 'Group 5'
      | sbobj.Groups.Signals(1).Name = 'mu'
      | sbobj.Groups.Signals(1).XData = [0 2 5 7 8.7 10.4 12.4 15 20]
      | sbobj.Groups.Signals(1).YData = [0 20.6 -19.5 -100 -120 -100 -40.1 -20 -10]
      | sbobj.Groups.Signals(2).Name = 'alpha'
      | sbobj.Groups.Signals(2).XData = [0 5 7.8 8.2 10 12.5 14 20]
      | sbobj.Groups.Signals(2).YData = [7 40 70 70 50 40.68 40 10]
      | sbobj.Groups.Signals(3).Name = 'beta'
      | sbobj.Groups.Signals(3).XData = [0 20]
      | sbobj.Groups.Signals(3).YData = [0 0]
      | sbobj.Groups.Signals(4).Name = 'speed brake'
      | sbobj.Groups.Signals(4).XData = [0 20]
      | sbobj.Groups.Signals(4).YData = [0 0]
      | sbobj.Groups.Signals(5).Name = 'LandingGear_down'
      | sbobj.Groups.Signals(5).XData = [0 20]
      | sbobj.Groups.Signals(5).YData = [1 1]
      | sbobj.Groups.TimeRange = [0 20]
  mu : Outport  Tag=STV Outport  VectorParamsAs1DForOutWhenUnconnected=off
  alpha : Outport  Tag=STV Outport  Port=2  VectorParamsAs1DForOutWhenUnconnected=off
  beta : Outport  Tag=STV Outport  Port=3  VectorParamsAs1DForOutWhenUnconnected=off
  speed brake : Outport  Tag=STV Outport  Port=4
  LandingGear_down : Outport  Tag=STV Outport  Port=5
  wires:
  FromWs/1 -> Demux/1
  Demux/1 -> mu/1
  Demux/2 -> alpha/1
  Demux/3 -> beta/1
  Demux/4 -> speed brake/1
  Demux/5 -> LandingGear_down/1

== system NDI/F-16 Vehicle Systems Model/Pilot commands storehouse/J trun(deg)0303meeting ==
  Demux : Demux  Tag=STV Demux  Outputs=5
      settings: DisplayOption=none
  FromWs : FromWorkspace  Tag=STV FromWs  VariableName=tuvar
      SigBuilderData=|
      | common.afterFinalStr = 'Extrapolate'
      | common.sampleTime = 0
      | dataSet.timeRange = [0 20]
      | dataSet.name = 'Group 5'
      | sbobj.Groups.Name = 'Group 5'
      | sbobj.Groups.Signals(1).Name = 'mu'
      | sbobj.Groups.Signals(1).XData = [0 2 5 6.5 8.2 9.5 11.4 11.4 15 20]
      | sbobj.Groups.Signals(1).YData = [0 26 -19.5 -100 -160 -100 -42 -40 -20 -10]
      | sbobj.Groups.Signals(2).Name = 'alpha'
      | sbobj.Groups.Signals(2).XData = [0 5 7.8 8.7 10 12.5 14 20]
      | sbobj.Groups.Signals(2).YData = [7 40 70 70 50 40.68 40 10]
      | sbobj.Groups.Signals(3).Name = 'beta'
      | sbobj.Groups.Signals(3).XData = [0 20]
      | sbobj.Groups.Signals(3).YData = [0 0]
      | sbobj.Groups.Signals(4).Name = 'speed brake'
      | sbobj.Groups.Signals(4).XData = [0 20]
      | sbobj.Groups.Signals(4).YData = [0 0]
      | sbobj.Groups.Signals(5).Name = 'LandingGear_down'
      | sbobj.Groups.Signals(5).XData = [0 20]
      | sbobj.Groups.Signals(5).YData = [1 1]
      | sbobj.Groups.TimeRange = [0 20]
  mu : Outport  Tag=STV Outport  VectorParamsAs1DForOutWhenUnconnected=off
  alpha : Outport  Tag=STV Outport  Port=2  VectorParamsAs1DForOutWhenUnconnected=off
  beta : Outport  Tag=STV Outport  Port=3  VectorParamsAs1DForOutWhenUnconnected=off
  speed brake : Outport  Tag=STV Outport  Port=4
  LandingGear_down : Outport  Tag=STV Outport  Port=5
  wires:
  FromWs/1 -> Demux/1
  Demux/1 -> mu/1
  Demux/2 -> alpha/1
  Demux/3 -> beta/1
  Demux/4 -> speed brake/1
  Demux/5 -> LandingGear_down/1

== system NDI/F-16 Vehicle Systems Model/Pilot commands storehouse/J trun(deg)0417meeting_1 ==
  Demux : Demux  Tag=STV Demux  Outputs=5
      settings: DisplayOption=none
  FromWs : FromWorkspace  Tag=STV FromWs  VariableName=tuvar
      SigBuilderData=|
      | common.afterFinalStr = 'Extrapolate'
      | common.sampleTime = 0
      | dataSet.timeRange = [0 20]
      | dataSet.name = 'Group 5'
      | sbobj.Groups.Name = 'Group 5'
      | sbobj.Groups.Signals(1).Name = 'mu'
      | sbobj.Groups.Signals(1).XData = [0 2 5 6.5 8.2 9.5 11.4 15 20]
      | sbobj.Groups.Signals(1).YData = [0 20.6 0 -100 -160 -100 -40.1 -20 -10]
      | sbobj.Groups.Signals(2).Name = 'alpha'
      | sbobj.Groups.Signals(2).XData = [0 5 7.8 9.5 11 12.5 14 20]
      | sbobj.Groups.Signals(2).YData = [7 40 70 70 50 40.68 40 10]
      | sbobj.Groups.Signals(3).Name = 'beta'
      | sbobj.Groups.Signals(3).XData = [0 20]
      | sbobj.Groups.Signals(3).YData = [0 0]
      | sbobj.Groups.Signals(4).Name = 'speed brake'
      | sbobj.Groups.Signals(4).XData = [0 20]
      | sbobj.Groups.Signals(4).YData = [0 0]
      | sbobj.Groups.Signals(5).Name = 'LandingGear_down'
      | sbobj.Groups.Signals(5).XData = [0 20]
      | sbobj.Groups.Signals(5).YData = [1 1]
      | sbobj.Groups.TimeRange = [0 20]
  mu : Outport  Tag=STV Outport  VectorParamsAs1DForOutWhenUnconnected=off
  alpha : Outport  Tag=STV Outport  Port=2  VectorParamsAs1DForOutWhenUnconnected=off
  beta : Outport  Tag=STV Outport  Port=3  VectorParamsAs1DForOutWhenUnconnected=off
  speed brake : Outport  Tag=STV Outport  Port=4
  LandingGear_down : Outport  Tag=STV Outport  Port=5
  wires:
  FromWs/1 -> Demux/1
  Demux/1 -> mu/1
  Demux/2 -> alpha/1
  Demux/3 -> beta/1
  Demux/4 -> speed brake/1
  Demux/5 -> LandingGear_down/1

== system NDI/F-16 Vehicle Systems Model/Pilot commands storehouse/J trun(deg)0417meeting_2 ==
  Demux : Demux  Tag=STV Demux  Outputs=5
      settings: DisplayOption=none
  FromWs : FromWorkspace  Tag=STV FromWs  VariableName=tuvar
      SigBuilderData=|
      | common.afterFinalStr = 'Extrapolate'
      | common.sampleTime = 0
      | dataSet.timeRange = [0 20]
      | dataSet.name = 'Group 5'
      | sbobj.Groups.Name = 'Group 5'
      | sbobj.Groups.Signals(1).Name = 'mu'
      | sbobj.Groups.Signals(1).XData = [0 2 5 6.5 8.2 9.5 11.4 15 20]
      | sbobj.Groups.Signals(1).YData = [0 20.6 0 -100 -160 -100 -40.1 -20 -10]
      | sbobj.Groups.Signals(2).Name = 'alpha'
      | sbobj.Groups.Signals(2).XData = [0 5 7.3 9.5 11 12.5 14 20]
      | sbobj.Groups.Signals(2).YData = [7 40 70 70 50 40.68 40 10]
      | sbobj.Groups.Signals(3).Name = 'beta'
      | sbobj.Groups.Signals(3).XData = [0 20]
      | sbobj.Groups.Signals(3).YData = [0 0]
      | sbobj.Groups.Signals(4).Name = 'speed brake'
      | sbobj.Groups.Signals(4).XData = [0 20]
      | sbobj.Groups.Signals(4).YData = [0 0]
      | sbobj.Groups.Signals(5).Name = 'LandingGear_down'
      | sbobj.Groups.Signals(5).XData = [0 20]
      | sbobj.Groups.Signals(5).YData = [1 1]
      | sbobj.Groups.TimeRange = [0 20]
  mu : Outport  Tag=STV Outport  VectorParamsAs1DForOutWhenUnconnected=off
  alpha : Outport  Tag=STV Outport  Port=2  VectorParamsAs1DForOutWhenUnconnected=off
  beta : Outport  Tag=STV Outport  Port=3  VectorParamsAs1DForOutWhenUnconnected=off
  speed brake : Outport  Tag=STV Outport  Port=4
  LandingGear_down : Outport  Tag=STV Outport  Port=5
  wires:
  FromWs/1 -> Demux/1
  Demux/1 -> mu/1
  Demux/2 -> alpha/1
  Demux/3 -> beta/1
  Demux/4 -> speed brake/1
  Demux/5 -> LandingGear_down/1

== system NDI/F-16 Vehicle Systems Model/Pilot commands storehouse/J trun(deg)0417meeting_3 ==
  Demux : Demux  Tag=STV Demux  Outputs=5
      settings: DisplayOption=none
  FromWs : FromWorkspace  Tag=STV FromWs  VariableName=tuvar
      SigBuilderData=|
      | common.afterFinalStr = 'Extrapolate'
      | common.sampleTime = 0
      | dataSet.timeRange = [0 20]
      | dataSet.name = 'Group 5'
      | sbobj.Groups.Name = 'Group 5'
      | sbobj.Groups.Signals(1).Name = 'mu'
      | sbobj.Groups.Signals(1).XData = [0 2 5 6.5 8.2 9.5 11.4 15 20]
      | sbobj.Groups.Signals(1).YData = [0 20.6 0 -100 -160 -100 -40.1 -20 -10]
      | sbobj.Groups.Signals(2).Name = 'alpha'
      | sbobj.Groups.Signals(2).XData = [0 5 6 9.5 11 12.5 14 20]
      | sbobj.Groups.Signals(2).YData = [7 40 70 70 50 40.68 40 10]
      | sbobj.Groups.Signals(3).Name = 'beta'
      | sbobj.Groups.Signals(3).XData = [0 20]
      | sbobj.Groups.Signals(3).YData = [0 0]
      | sbobj.Groups.Signals(4).Name = 'speed brake'
      | sbobj.Groups.Signals(4).XData = [0 20]
      | sbobj.Groups.Signals(4).YData = [0 0]
      | sbobj.Groups.Signals(5).Name = 'LandingGear_down'
      | sbobj.Groups.Signals(5).XData = [0 20]
      | sbobj.Groups.Signals(5).YData = [1 1]
      | sbobj.Groups.TimeRange = [0 20]
  mu : Outport  Tag=STV Outport  VectorParamsAs1DForOutWhenUnconnected=off
  alpha : Outport  Tag=STV Outport  Port=2  VectorParamsAs1DForOutWhenUnconnected=off
  beta : Outport  Tag=STV Outport  Port=3  VectorParamsAs1DForOutWhenUnconnected=off
  speed brake : Outport  Tag=STV Outport  Port=4
  LandingGear_down : Outport  Tag=STV Outport  Port=5
  wires:
  FromWs/1 -> Demux/1
  Demux/1 -> mu/1
  Demux/2 -> alpha/1
  Demux/3 -> beta/1
  Demux/4 -> speed brake/1
  Demux/5 -> LandingGear_down/1

== system NDI/F-16 Vehicle Systems Model/Pilot commands storehouse/J trun(deg)0417meeting_4 ==
  Demux : Demux  Tag=STV Demux  Outputs=5
      settings: DisplayOption=none
  FromWs : FromWorkspace  Tag=STV FromWs  VariableName=tuvar
      SigBuilderData=|
      | common.afterFinalStr = 'Extrapolate'
      | common.sampleTime = 0
      | dataSet.timeRange = [0 20]
      | dataSet.name = 'Group 5'
      | sbobj.Groups.Name = 'Group 5'
      | sbobj.Groups.Signals(1).Name = 'mu'
      | sbobj.Groups.Signals(1).XData = [0 2 5 6.5 8.2 9.5 11.4 15 20]
      | sbobj.Groups.Signals(1).YData = [0 20.6 0 -100 -160 -100 -40.1 -20 -10]
      | sbobj.Groups.Signals(2).Name = 'alpha'
      | sbobj.Groups.Signals(2).XData = [0 5 6 9.5 11 12.5 14 20]
      | sbobj.Groups.Signals(2).YData = [7 40 80 80 50 40.68 40 10]
      | sbobj.Groups.Signals(3).Name = 'beta'
      | sbobj.Groups.Signals(3).XData = [0 20]
      | sbobj.Groups.Signals(3).YData = [0 0]
      | sbobj.Groups.Signals(4).Name = 'speed brake'
      | sbobj.Groups.Signals(4).XData = [0 20]
      | sbobj.Groups.Signals(4).YData = [0 0]
      | sbobj.Groups.Signals(5).Name = 'LandingGear_down'
      | sbobj.Groups.Signals(5).XData = [0 20]
      | sbobj.Groups.Signals(5).YData = [1 1]
      | sbobj.Groups.TimeRange = [0 20]
  mu : Outport  Tag=STV Outport  VectorParamsAs1DForOutWhenUnconnected=off
  alpha : Outport  Tag=STV Outport  Port=2  VectorParamsAs1DForOutWhenUnconnected=off
  beta : Outport  Tag=STV Outport  Port=3  VectorParamsAs1DForOutWhenUnconnected=off
  speed brake : Outport  Tag=STV Outport  Port=4
  LandingGear_down : Outport  Tag=STV Outport  Port=5
  wires:
  FromWs/1 -> Demux/1
  Demux/1 -> mu/1
  Demux/2 -> alpha/1
  Demux/3 -> beta/1
  Demux/4 -> speed brake/1
  Demux/5 -> LandingGear_down/1

== system NDI/F-16 Vehicle Systems Model/Pilot commands storehouse/J trun(deg)0417meeting_5 ==
  Demux : Demux  Tag=STV Demux  Outputs=5
      settings: DisplayOption=none
  FromWs : FromWorkspace  Tag=STV FromWs  VariableName=tuvar
      SigBuilderData=|
      | common.afterFinalStr = 'Extrapolate'
      | common.sampleTime = 0
      | dataSet.timeRange = [0 20]
      | dataSet.name = 'Group 5'
      | sbobj.Groups.Name = 'Group 5'
      | sbobj.Groups.Signals(1).Name = 'mu'
      | sbobj.Groups.Signals(1).XData = [0 2 5 6.5 8.2 9.5 11.4 15 20]
      | sbobj.Groups.Signals(1).YData = [0 20.6 0 -100 -170 -100 -40.1 -20 -10]
      | sbobj.Groups.Signals(2).Name = 'alpha'
      | sbobj.Groups.Signals(2).XData = [0 5 6 9.5 11 12.5 14 20]
      | sbobj.Groups.Signals(2).YData = [7 40 90 90 50 40.68 40 10]
      | sbobj.Groups.Signals(3).Name = 'beta'
      | sbobj.Groups.Signals(3).XData = [0 20]
      | sbobj.Groups.Signals(3).YData = [0 0]
      | sbobj.Groups.Signals(4).Name = 'speed brake'
      | sbobj.Groups.Signals(4).XData = [0 20]
      | sbobj.Groups.Signals(4).YData = [0 0]
      | sbobj.Groups.Signals(5).Name = 'LandingGear_down'
      | sbobj.Groups.Signals(5).XData = [0 20]
      | sbobj.Groups.Signals(5).YData = [1 1]
      | sbobj.Groups.TimeRange = [0 20]
  mu : Outport  Tag=STV Outport  VectorParamsAs1DForOutWhenUnconnected=off
  alpha : Outport  Tag=STV Outport  Port=2  VectorParamsAs1DForOutWhenUnconnected=off
  beta : Outport  Tag=STV Outport  Port=3  VectorParamsAs1DForOutWhenUnconnected=off
  speed brake : Outport  Tag=STV Outport  Port=4
  LandingGear_down : Outport  Tag=STV Outport  Port=5
  wires:
  FromWs/1 -> Demux/1
  Demux/1 -> mu/1
  Demux/2 -> alpha/1
  Demux/3 -> beta/1
  Demux/4 -> speed brake/1
  Demux/5 -> LandingGear_down/1

== system NDI/F-16 Vehicle Systems Model/Pilot commands storehouse/J trun(deg)初始高度6560ft 初始速度250ft//s(碩論6.4,6.5) ==
  Demux : Demux  Tag=STV Demux  Outputs=5
      settings: DisplayOption=none
  FromWs : FromWorkspace  Tag=STV FromWs  VariableName=tuvar
      SigBuilderData=|
      | common.afterFinalStr = 'Extrapolate'
      | common.sampleTime = 0
      | dataSet.timeRange = [0 20]
      | dataSet.name = 'Group 5'
      | sbobj.Groups.Name = 'Group 5'
      | sbobj.Groups.Signals(1).Name = 'mu'
      | sbobj.Groups.Signals(1).XData = [0 2 5 6.5 8.2 9.5 11.4 15 20]
      | sbobj.Groups.Signals(1).YData = [0 26 -19.5 -100 -160 -105 -80 -47.5 -10]
      | sbobj.Groups.Signals(2).Name = 'alpha'
      | sbobj.Groups.Signals(2).XData = [0 5 7.8 8.7 10 12.5 14 20]
      | sbobj.Groups.Signals(2).YData = [7 40 70 70 50 40.68 40 10]
      | sbobj.Groups.Signals(3).Name = 'beta'
      | sbobj.Groups.Signals(3).XData = [0 20]
      | sbobj.Groups.Signals(3).YData = [0 0]
      | sbobj.Groups.Signals(4).Name = 'speed brake'
      | sbobj.Groups.Signals(4).XData = [0 20]
      | sbobj.Groups.Signals(4).YData = [0 0]
      | sbobj.Groups.Signals(5).Name = 'LandingGear_down'
      | sbobj.Groups.Signals(5).XData = [0 20]
      | sbobj.Groups.Signals(5).YData = [1 1]
      | sbobj.Groups.TimeRange = [0 20]
  mu : Outport  Tag=STV Outport  VectorParamsAs1DForOutWhenUnconnected=off
  alpha : Outport  Tag=STV Outport  Port=2  VectorParamsAs1DForOutWhenUnconnected=off
  beta : Outport  Tag=STV Outport  Port=3  VectorParamsAs1DForOutWhenUnconnected=off
  speed brake : Outport  Tag=STV Outport  Port=4
  LandingGear_down : Outport  Tag=STV Outport  Port=5
  wires:
  FromWs/1 -> Demux/1
  Demux/1 -> mu/1
  Demux/2 -> alpha/1
  Demux/3 -> beta/1
  Demux/4 -> speed brake/1
  Demux/5 -> LandingGear_down/1

== system NDI/F-16 Vehicle Systems Model/Pilot commands storehouse/J trun(deg)初始高度6560ft 初始速度250ft//s(碩論6.6,6.8.2,7.2) ==
  Demux : Demux  Tag=STV Demux  Outputs=5
      settings: DisplayOption=none
  FromWs : FromWorkspace  Tag=STV FromWs  VariableName=tuvar
      SigBuilderData=|
      | common.afterFinalStr = 'Extrapolate'
      | common.sampleTime = 0
      | dataSet.timeRange = [0 20]
      | dataSet.name = 'Group 5'
      | sbobj.Groups.Name = 'Group 5'
      | sbobj.Groups.Signals(1).Name = 'mu'
      | sbobj.Groups.Signals(1).XData = [0 2 5 6.5 8.2 9.5 11.4 15 20]
      | sbobj.Groups.Signals(1).YData = [0 26 -19.5 -100 -160 -105 -80 -60 -10]
      | sbobj.Groups.Signals(2).Name = 'alpha'
      | sbobj.Groups.Signals(2).XData = [0 5 7.8 8.7 10 12.5 14 20]
      | sbobj.Groups.Signals(2).YData = [7 40 80 80 50 40.68 40 10]
      | sbobj.Groups.Signals(3).Name = 'beta'
      | sbobj.Groups.Signals(3).XData = [0 20]
      | sbobj.Groups.Signals(3).YData = [0 0]
      | sbobj.Groups.Signals(4).Name = 'speed brake'
      | sbobj.Groups.Signals(4).XData = [0 20]
      | sbobj.Groups.Signals(4).YData = [0 0]
      | sbobj.Groups.Signals(5).Name = 'LandingGear_down'
      | sbobj.Groups.Signals(5).XData = [0 20]
      | sbobj.Groups.Signals(5).YData = [1 1]
      | sbobj.Groups.TimeRange = [0 20]
  mu : Outport  Tag=STV Outport  VectorParamsAs1DForOutWhenUnconnected=off
  alpha : Outport  Tag=STV Outport  Port=2  VectorParamsAs1DForOutWhenUnconnected=off
  beta : Outport  Tag=STV Outport  Port=3  VectorParamsAs1DForOutWhenUnconnected=off
  speed brake : Outport  Tag=STV Outport  Port=4
  LandingGear_down : Outport  Tag=STV Outport  Port=5
  wires:
  FromWs/1 -> Demux/1
  Demux/1 -> mu/1
  Demux/2 -> alpha/1
  Demux/3 -> beta/1
  Demux/4 -> speed brake/1
  Demux/5 -> LandingGear_down/1

== system NDI/F-16 Vehicle Systems Model/Pilot commands storehouse/J trun(deg)初始高度6560ft 初始速度250ft//s(碩論6.8.2)更正 ==
  Demux : Demux  Tag=STV Demux  Outputs=5
      settings: DisplayOption=none
  FromWs : FromWorkspace  Tag=STV FromWs  VariableName=tuvar
      SigBuilderData=|
      | common.afterFinalStr = 'Extrapolate'
      | common.sampleTime = 0
      | dataSet.timeRange = [0 20]
      | dataSet.name = 'Group 5'
      | sbobj.Groups.Name = 'Group 5'
      | sbobj.Groups.Signals(1).Name = 'mu'
      | sbobj.Groups.Signals(1).XData = [0 2 5 6.5 8.2 9.3 11.4 15 20]
      | sbobj.Groups.Signals(1).YData = [0 26 -19.5 -110 -170 -105 -90 -80 -60]
      | sbobj.Groups.Signals(2).Name = 'alpha'
      | sbobj.Groups.Signals(2).XData = [0 5 7.8 8.7 10 12.5 14 20]
      | sbobj.Groups.Signals(2).YData = [7 40 80 80 50 40.68 40 10]
      | sbobj.Groups.Signals(3).Name = 'beta'
      | sbobj.Groups.Signals(3).XData = [0 20]
      | sbobj.Groups.Signals(3).YData = [0 0]
      | sbobj.Groups.Signals(4).Name = 'speed brake'
      | sbobj.Groups.Signals(4).XData = [0 20]
      | sbobj.Groups.Signals(4).YData = [0 0]
      | sbobj.Groups.Signals(5).Name = 'LandingGear_down'
      | sbobj.Groups.Signals(5).XData = [0 20]
      | sbobj.Groups.Signals(5).YData = [1 1]
      | sbobj.Groups.TimeRange = [0 20]
  mu : Outport  Tag=STV Outport  VectorParamsAs1DForOutWhenUnconnected=off
  alpha : Outport  Tag=STV Outport  Port=2  VectorParamsAs1DForOutWhenUnconnected=off
  beta : Outport  Tag=STV Outport  Port=3  VectorParamsAs1DForOutWhenUnconnected=off
  speed brake : Outport  Tag=STV Outport  Port=4
  LandingGear_down : Outport  Tag=STV Outport  Port=5
  wires:
  FromWs/1 -> Demux/1
  Demux/1 -> mu/1
  Demux/2 -> alpha/1
  Demux/3 -> beta/1
  Demux/4 -> speed brake/1
  Demux/5 -> LandingGear_down/1

== system NDI/F-16 Vehicle Systems Model/Pilot commands storehouse/J trun(rad) ==
  Demux : Demux  Tag=STV Demux  Outputs=5
      settings: DisplayOption=none
  FromWs : FromWorkspace  Tag=STV FromWs  VariableName=tuvar
      SigBuilderData=|
      | common.afterFinalStr = 'Extrapolate'
      | common.sampleTime = 0
      | dataSet.timeRange = [0 20]
      | dataSet.name = 'Group 5'
      | sbobj.Groups.Name = 'Group 5'
      | sbobj.Groups.Signals(1).Name = 'mu'
      | sbobj.Groups.Signals(1).XData = [0 2 5 7 8.7 8.7 10.4 12.4 15 20]
      | sbobj.Groups.Signals(1).YData = [0 0.36 -0.34 -1.74 -2.09 -2.1 -1.74 -0.7 -0.349 -0.174]
      | sbobj.Groups.Signals(2).Name = 'alpha'
      | sbobj.Groups.Signals(2).XData = [0 5 7.8 8.2 10 12.5 14 20]
      | sbobj.Groups.Signals(2).YData = [0.122 0.698 1.2 1.2 0.87 0.71 0.698 0.1745]
      | sbobj.Groups.Signals(3).Name = 'beta'
      | sbobj.Groups.Signals(3).XData = [0 20]
      | sbobj.Groups.Signals(3).YData = [0 0]
      | sbobj.Groups.Signals(4).Name = 'speed brake'
      | sbobj.Groups.Signals(4).XData = [0 20]
      | sbobj.Groups.Signals(4).YData = [0 0]
      | sbobj.Groups.Signals(5).Name = 'LandingGear_down'
      | sbobj.Groups.Signals(5).XData = [0 20]
      | sbobj.Groups.Signals(5).YData = [1 1]
      | sbobj.Groups.TimeRange = [0 20]
  mu : Outport  Tag=STV Outport  VectorParamsAs1DForOutWhenUnconnected=off
  alpha : Outport  Tag=STV Outport  Port=2  VectorParamsAs1DForOutWhenUnconnected=off
  beta : Outport  Tag=STV Outport  Port=3  VectorParamsAs1DForOutWhenUnconnected=off
  speed brake : Outport  Tag=STV Outport  Port=4
  LandingGear_down : Outport  Tag=STV Outport  Port=5
  wires:
  FromWs/1 -> Demux/1
  Demux/1 -> mu/1
  Demux/2 -> alpha/1
  Demux/3 -> beta/1
  Demux/4 -> speed brake/1
  Demux/5 -> LandingGear_down/1

== system NDI/F-16 Vehicle Systems Model/Pilot commands storehouse/trun(deg) 初始高度10000ft 初始速度100ft//s攻角30度 ==
  Demux : Demux  Tag=STV Demux  Outputs=5
      settings: DisplayOption=none
  FromWs : FromWorkspace  Tag=STV FromWs  VariableName=tuvar
      SigBuilderData=|
      | common.afterFinalStr = 'Extrapolate'
      | common.sampleTime = 0
      | dataSet.timeRange = [0 20]
      | dataSet.name = 'Group 5'
      | sbobj.Groups.Name = 'Group 5'
      | sbobj.Groups.Signals(1).Name = 'mu'
      | sbobj.Groups.Signals(1).XData = [0 2 5.5 6.5 8.2 9.5 10 13 15 20]
      | sbobj.Groups.Signals(1).YData = [0 0 0 -80 -120 -120 -120 -70 -40 -10]
      | sbobj.Groups.Signals(2).Name = 'alpha'
      | sbobj.Groups.Signals(2).XData = [0 4 7.8 9.2 12.5 14 16 20]
      | sbobj.Groups.Signals(2).YData = [5 5 30 30 10 5 5 5]
      | sbobj.Groups.Signals(3).Name = 'beta'
      | sbobj.Groups.Signals(3).XData = [0 20]
      | sbobj.Groups.Signals(3).YData = [0 0]
      | sbobj.Groups.Signals(4).Name = 'speed brake'
      | sbobj.Groups.Signals(4).XData = [0 20]
      | sbobj.Groups.Signals(4).YData = [0 0]
      | sbobj.Groups.Signals(5).Name = 'LandingGear_down'
      | sbobj.Groups.Signals(5).XData = [0 20]
      | sbobj.Groups.Signals(5).YData = [1 1]
      | sbobj.Groups.TimeRange = [0 20]
  mu : Outport  Tag=STV Outport  VectorParamsAs1DForOutWhenUnconnected=off
  alpha : Outport  Tag=STV Outport  Port=2  VectorParamsAs1DForOutWhenUnconnected=off
  beta : Outport  Tag=STV Outport  Port=3  VectorParamsAs1DForOutWhenUnconnected=off
  speed brake : Outport  Tag=STV Outport  Port=4
  LandingGear_down : Outport  Tag=STV Outport  Port=5
  wires:
  Demux/5 -> LandingGear_down/1
  Demux/4 -> speed brake/1
  Demux/3 -> beta/1
  Demux/2 -> alpha/1
  Demux/1 -> mu/1
  FromWs/1 -> Demux/1

== system NDI/F-16 Vehicle Systems Model/Pilot commands storehouse/trun(deg) 初始高度10000ft 初始速度150ft//s攻角40度1 ==
  Demux : Demux  Tag=STV Demux  Outputs=5
      settings: DisplayOption=none
  FromWs : FromWorkspace  Tag=STV FromWs  VariableName=tuvar
      SigBuilderData=|
      | common.afterFinalStr = 'Extrapolate'
      | common.sampleTime = 0
      | dataSet.timeRange = [0 20]
      | dataSet.name = 'Group 5'
      | sbobj.Groups.Name = 'Group 5'
      | sbobj.Groups.Signals(1).Name = 'mu'
      | sbobj.Groups.Signals(1).XData = [0 2 5.5 7 8.7 10 11 13 15 20]
      | sbobj.Groups.Signals(1).YData = [0 0 -19.5 -60 -150 -150 -150 -70 -40 -10]
      | sbobj.Groups.Signals(2).Name = 'alpha'
      | sbobj.Groups.Signals(2).XData = [0 5 7.8 8.2 10 12.5 14 20]
      | sbobj.Groups.Signals(2).YData = [7 10 40 40 20 10.68 10 10]
      | sbobj.Groups.Signals(3).Name = 'beta'
      | sbobj.Groups.Signals(3).XData = [0 20]
      | sbobj.Groups.Signals(3).YData = [0 0]
      | sbobj.Groups.Signals(4).Name = 'speed brake'
      | sbobj.Groups.Signals(4).XData = [0 20]
      | sbobj.Groups.Signals(4).YData = [0 0]
      | sbobj.Groups.Signals(5).Name = 'LandingGear_down'
      | sbobj.Groups.Signals(5).XData = [0 20]
      | sbobj.Groups.Signals(5).YData = [1 1]
      | sbobj.Groups.TimeRange = [0 20]
  mu : Outport  Tag=STV Outport  VectorParamsAs1DForOutWhenUnconnected=off
  alpha : Outport  Tag=STV Outport  Port=2  VectorParamsAs1DForOutWhenUnconnected=off
  beta : Outport  Tag=STV Outport  Port=3  VectorParamsAs1DForOutWhenUnconnected=off
  speed brake : Outport  Tag=STV Outport  Port=4
  LandingGear_down : Outport  Tag=STV Outport  Port=5
  wires:
  Demux/5 -> LandingGear_down/1
  Demux/4 -> speed brake/1
  Demux/3 -> beta/1
  Demux/2 -> alpha/1
  Demux/1 -> mu/1
  FromWs/1 -> Demux/1

== system NDI/F-16 Vehicle Systems Model/Pilot commands storehouse/trun(deg) 初始高度10000ft 初始速度250ft//s攻角40度1 ==
  Demux : Demux  Tag=STV Demux  Outputs=5
      settings: DisplayOption=none
  FromWs : FromWorkspace  Tag=STV FromWs  VariableName=tuvar
      SigBuilderData=|
      | common.afterFinalStr = 'Extrapolate'
      | common.sampleTime = 0
      | dataSet.timeRange = [0 20]
      | dataSet.name = 'Group 5'
      | sbobj.Groups.Name = 'Group 5'
      | sbobj.Groups.Signals(1).Name = 'mu'
      | sbobj.Groups.Signals(1).XData = [0 2 5.5 7 8.7 8.7 10 11 13 15 20]
      | sbobj.Groups.Signals(1).YData = [0 0 -19.5 -122 -172 -170 -170 -170 -70 -40 -10]
      | sbobj.Groups.Signals(2).Name = 'alpha'
      | sbobj.Groups.Signals(2).XData = [0 5 7.8 8.2 10 12.5 14 20]
      | sbobj.Groups.Signals(2).YData = [7 10 40 40 20 10.68 10 10]
      | sbobj.Groups.Signals(3).Name = 'beta'
      | sbobj.Groups.Signals(3).XData = [0 20]
      | sbobj.Groups.Signals(3).YData = [0 0]
      | sbobj.Groups.Signals(4).Name = 'speed brake'
      | sbobj.Groups.Signals(4).XData = [0 20]
      | sbobj.Groups.Signals(4).YData = [0 0]
      | sbobj.Groups.Signals(5).Name = 'LandingGear_down'
      | sbobj.Groups.Signals(5).XData = [0 20]
      | sbobj.Groups.Signals(5).YData = [1 1]
      | sbobj.Groups.TimeRange = [0 20]
  mu : Outport  Tag=STV Outport  VectorParamsAs1DForOutWhenUnconnected=off
  alpha : Outport  Tag=STV Outport  Port=2  VectorParamsAs1DForOutWhenUnconnected=off
  beta : Outport  Tag=STV Outport  Port=3  VectorParamsAs1DForOutWhenUnconnected=off
  speed brake : Outport  Tag=STV Outport  Port=4
  LandingGear_down : Outport  Tag=STV Outport  Port=5
  wires:
  Demux/5 -> LandingGear_down/1
  Demux/4 -> speed brake/1
  Demux/3 -> beta/1
  Demux/2 -> alpha/1
  Demux/1 -> mu/1
  FromWs/1 -> Demux/1

== system NDI/F-16 Vehicle Systems Model/Pilot commands storehouse/trun(deg) 初始高度10000ft 初始速度350ft//s攻角40度 ==
  Demux : Demux  Tag=STV Demux  Outputs=5
      settings: DisplayOption=none
  FromWs : FromWorkspace  Tag=STV FromWs  VariableName=tuvar
      SigBuilderData=|
      | common.afterFinalStr = 'Extrapolate'
      | common.sampleTime = 0
      | dataSet.timeRange = [0 20]
      | dataSet.name = 'Group 5'
      | sbobj.Groups.Name = 'Group 5'
      | sbobj.Groups.Signals(1).Name = 'mu'
      | sbobj.Groups.Signals(1).XData = [0 2 5.5 6.5 8.2 10 11 13 15 20]
      | sbobj.Groups.Signals(1).YData = [0 0 -19.5 -122 -170 -170 -170 -70 -40 -10]
      | sbobj.Groups.Signals(2).Name = 'alpha'
      | sbobj.Groups.Signals(2).XData = [0 5 7.8 8.2 10 12.5 14 20]
      | sbobj.Groups.Signals(2).YData = [7 10 40 40 20 10.68 10 10]
      | sbobj.Groups.Signals(3).Name = 'beta'
      | sbobj.Groups.Signals(3).XData = [0 20]
      | sbobj.Groups.Signals(3).YData = [0 0]
      | sbobj.Groups.Signals(4).Name = 'speed brake'
      | sbobj.Groups.Signals(4).XData = [0 20]
      | sbobj.Groups.Signals(4).YData = [0 0]
      | sbobj.Groups.Signals(5).Name = 'LandingGear_down'
      | sbobj.Groups.Signals(5).XData = [0 20]
      | sbobj.Groups.Signals(5).YData = [1 1]
      | sbobj.Groups.TimeRange = [0 20]
  mu : Outport  Tag=STV Outport  VectorParamsAs1DForOutWhenUnconnected=off
  alpha : Outport  Tag=STV Outport  Port=2  VectorParamsAs1DForOutWhenUnconnected=off
  beta : Outport  Tag=STV Outport  Port=3  VectorParamsAs1DForOutWhenUnconnected=off
  speed brake : Outport  Tag=STV Outport  Port=4
  LandingGear_down : Outport  Tag=STV Outport  Port=5
  wires:
  Demux/5 -> LandingGear_down/1
  Demux/4 -> speed brake/1
  Demux/3 -> beta/1
  Demux/2 -> alpha/1
  Demux/1 -> mu/1
  FromWs/1 -> Demux/1

== system NDI/F-16 Vehicle Systems Model/Pilot commands storehouse/trun(deg) 初始高度10000ft 初始速度450ft//s攻角40度 ==
  Demux : Demux  Tag=STV Demux  Outputs=5
      settings: DisplayOption=none
  FromWs : FromWorkspace  Tag=STV FromWs  VariableName=tuvar
      SigBuilderData=|
      | common.afterFinalStr = 'Extrapolate'
      | common.sampleTime = 0
      | dataSet.timeRange = [0 20]
      | dataSet.name = 'Group 5'
      | sbobj.Groups.Name = 'Group 5'
      | sbobj.Groups.Signals(1).Name = 'mu'
      | sbobj.Groups.Signals(1).XData = [0 2 5.5 6.5 7.5 8.5 10 12 15 20]
      | sbobj.Groups.Signals(1).YData = [0 0 -19.5 -120 -150 -150 -150 -70 -40 -10]
      | sbobj.Groups.Signals(2).Name = 'alpha'
      | sbobj.Groups.Signals(2).XData = [0 5 7.2 7.8 10 12.5 14 20]
      | sbobj.Groups.Signals(2).YData = [7 10 40 40 20 10.68 10 10]
      | sbobj.Groups.Signals(3).Name = 'beta'
      | sbobj.Groups.Signals(3).XData = [0 20]
      | sbobj.Groups.Signals(3).YData = [0 0]
      | sbobj.Groups.Signals(4).Name = 'speed brake'
      | sbobj.Groups.Signals(4).XData = [0 20]
      | sbobj.Groups.Signals(4).YData = [0 0]
      | sbobj.Groups.Signals(5).Name = 'LandingGear_down'
      | sbobj.Groups.Signals(5).XData = [0 20]
      | sbobj.Groups.Signals(5).YData = [1 1]
      | sbobj.Groups.TimeRange = [0 20]
  mu : Outport  Tag=STV Outport  VectorParamsAs1DForOutWhenUnconnected=off
  alpha : Outport  Tag=STV Outport  Port=2  VectorParamsAs1DForOutWhenUnconnected=off
  beta : Outport  Tag=STV Outport  Port=3  VectorParamsAs1DForOutWhenUnconnected=off
  speed brake : Outport  Tag=STV Outport  Port=4
  LandingGear_down : Outport  Tag=STV Outport  Port=5
  wires:
  Demux/5 -> LandingGear_down/1
  Demux/4 -> speed brake/1
  Demux/3 -> beta/1
  Demux/2 -> alpha/1
  Demux/1 -> mu/1
  FromWs/1 -> Demux/1

== system NDI/F-16 Vehicle Systems Model/Pilot commands storehouse/trun(deg) 初始高度10000ft 初始速度450ft//s攻角40度1 ==
  Demux : Demux  Tag=STV Demux  Outputs=5
      settings: DisplayOption=none
  FromWs : FromWorkspace  Tag=STV FromWs  VariableName=tuvar
      SigBuilderData=|
      | common.afterFinalStr = 'Extrapolate'
      | common.sampleTime = 0
      | dataSet.timeRange = [0 20]
      | dataSet.name = 'Group 5'
      | sbobj.Groups.Name = 'Group 5'
      | sbobj.Groups.Signals(1).Name = 'mu'
      | sbobj.Groups.Signals(1).XData = [0 2 5.5 6.5 7.5 8.5 10 12 15 20]
      | sbobj.Groups.Signals(1).YData = [0 0 -19.5 -120 -150 -150 -150 -70 -40 -10]
      | sbobj.Groups.Signals(2).Name = 'alpha'
      | sbobj.Groups.Signals(2).XData = [0 5 7.2 7.8 10 12.5 14 20]
      | sbobj.Groups.Signals(2).YData = [7 10 40 40 20 10.68 10 10]
      | sbobj.Groups.Signals(3).Name = 'beta'
      | sbobj.Groups.Signals(3).XData = [0 20]
      | sbobj.Groups.Signals(3).YData = [0 0]
      | sbobj.Groups.Signals(4).Name = 'speed brake'
      | sbobj.Groups.Signals(4).XData = [0 20]
      | sbobj.Groups.Signals(4).YData = [0 0]
      | sbobj.Groups.Signals(5).Name = 'LandingGear_down'
      | sbobj.Groups.Signals(5).XData = [0 20]
      | sbobj.Groups.Signals(5).YData = [1 1]
      | sbobj.Groups.TimeRange = [0 20]
  mu : Outport  Tag=STV Outport  VectorParamsAs1DForOutWhenUnconnected=off
  alpha : Outport  Tag=STV Outport  Port=2  VectorParamsAs1DForOutWhenUnconnected=off
  beta : Outport  Tag=STV Outport  Port=3  VectorParamsAs1DForOutWhenUnconnected=off
  speed brake : Outport  Tag=STV Outport  Port=4
  LandingGear_down : Outport  Tag=STV Outport  Port=5
  wires:
  Demux/5 -> LandingGear_down/1
  Demux/4 -> speed brake/1
  Demux/3 -> beta/1
  Demux/2 -> alpha/1
  Demux/1 -> mu/1
  FromWs/1 -> Demux/1

== system NDI/F-16 Vehicle Systems Model/Pilot commands storehouse/trun(deg) 初始高度10000ft 初始速度500ft//s攻角30度1 ==
  Demux : Demux  Tag=STV Demux  Outputs=5
      settings: DisplayOption=none
  FromWs : FromWorkspace  Tag=STV FromWs  VariableName=tuvar
      SigBuilderData=|
      | common.afterFinalStr = 'Extrapolate'
      | common.sampleTime = 0
      | dataSet.timeRange = [0 20]
      | dataSet.name = 'Group 5'
      | sbobj.Groups.Name = 'Group 5'
      | sbobj.Groups.Signals(1).Name = 'mu'
      | sbobj.Groups.Signals(1).XData = [0 2 5.5 6.7 8.2 9.5 10 13 15 20]
      | sbobj.Groups.Signals(1).YData = [0 0 20 -80 -120 -120 -120 -70 -40 -10]
      | sbobj.Groups.Signals(2).Name = 'alpha'
      | sbobj.Groups.Signals(2).XData = [0 2 5.8 9.2 12.5 14 16 20]
      | sbobj.Groups.Signals(2).YData = [5 5 30 30 10 5 5 5]
      | sbobj.Groups.Signals(3).Name = 'beta'
      | sbobj.Groups.Signals(3).XData = [0 20]
      | sbobj.Groups.Signals(3).YData = [0 0]
      | sbobj.Groups.Signals(4).Name = 'speed brake'
      | sbobj.Groups.Signals(4).XData = [0 20]
      | sbobj.Groups.Signals(4).YData = [0 0]
      | sbobj.Groups.Signals(5).Name = 'LandingGear_down'
      | sbobj.Groups.Signals(5).XData = [0 20]
      | sbobj.Groups.Signals(5).YData = [1 1]
      | sbobj.Groups.TimeRange = [0 20]
  mu : Outport  Tag=STV Outport  VectorParamsAs1DForOutWhenUnconnected=off
  alpha : Outport  Tag=STV Outport  Port=2  VectorParamsAs1DForOutWhenUnconnected=off
  beta : Outport  Tag=STV Outport  Port=3  VectorParamsAs1DForOutWhenUnconnected=off
  speed brake : Outport  Tag=STV Outport  Port=4
  LandingGear_down : Outport  Tag=STV Outport  Port=5
  wires:
  Demux/5 -> LandingGear_down/1
  Demux/4 -> speed brake/1
  Demux/3 -> beta/1
  Demux/2 -> alpha/1
  Demux/1 -> mu/1
  FromWs/1 -> Demux/1

== system NDI/F-16 Vehicle Systems Model/Pilot commands storehouse/trun(deg) 初始高度10000ft 初始速度550ft//s攻角40度 ==
  Demux : Demux  Tag=STV Demux  Outputs=5
      settings: DisplayOption=none
  FromWs : FromWorkspace  Tag=STV FromWs  VariableName=tuvar
      SigBuilderData=|
      | common.afterFinalStr = 'Extrapolate'
      | common.sampleTime = 0
      | dataSet.timeRange = [0 20]
      | dataSet.name = 'Group 5'
      | sbobj.Groups.Name = 'Group 5'
      | sbobj.Groups.Signals(1).Name = 'mu'
      | sbobj.Groups.Signals(1).XData = [0 2 5.5 6 7.2 8.5 10 12 15 20]
      | sbobj.Groups.Signals(1).YData = [0 0 -19.5 -120 -150 -150 -150 -70 -40 -10]
      | sbobj.Groups.Signals(2).Name = 'alpha'
      | sbobj.Groups.Signals(2).XData = [0 5 7.2 7.8 10 12.5 14 20]
      | sbobj.Groups.Signals(2).YData = [7 10 40 40 20 10.68 10 10]
      | sbobj.Groups.Signals(3).Name = 'beta'
      | sbobj.Groups.Signals(3).XData = [0 20]
      | sbobj.Groups.Signals(3).YData = [0 0]
      | sbobj.Groups.Signals(4).Name = 'speed brake'
      | sbobj.Groups.Signals(4).XData = [0 20]
      | sbobj.Groups.Signals(4).YData = [0 0]
      | sbobj.Groups.Signals(5).Name = 'LandingGear_down'
      | sbobj.Groups.Signals(5).XData = [0 20]
      | sbobj.Groups.Signals(5).YData = [1 1]
      | sbobj.Groups.TimeRange = [0 20]
  mu : Outport  Tag=STV Outport  VectorParamsAs1DForOutWhenUnconnected=off
  alpha : Outport  Tag=STV Outport  Port=2  VectorParamsAs1DForOutWhenUnconnected=off
  beta : Outport  Tag=STV Outport  Port=3  VectorParamsAs1DForOutWhenUnconnected=off
  speed brake : Outport  Tag=STV Outport  Port=4
  LandingGear_down : Outport  Tag=STV Outport  Port=5
  wires:
  Demux/5 -> LandingGear_down/1
  Demux/4 -> speed brake/1
  Demux/3 -> beta/1
  Demux/2 -> alpha/1
  Demux/1 -> mu/1
  FromWs/1 -> Demux/1

== system NDI/F-16 Vehicle Systems Model/Pilot commands storehouse/trun(deg) 初始高度10000ft 初始速度550ft//s攻角40度1 ==
  Demux : Demux  Tag=STV Demux  Outputs=5
      settings: DisplayOption=none
  FromWs : FromWorkspace  Tag=STV FromWs  VariableName=tuvar
      SigBuilderData=|
      | common.afterFinalStr = 'Extrapolate'
      | common.sampleTime = 0
      | dataSet.timeRange = [0 20]
      | dataSet.name = 'Group 5'
      | sbobj.Groups.Name = 'Group 5'
      | sbobj.Groups.Signals(1).Name = 'mu'
      | sbobj.Groups.Signals(1).XData = [0 2 5.5 6 7.2 8.5 10 12 15 20]
      | sbobj.Groups.Signals(1).YData = [0 0 -19.5 -120 -150 -150 -150 -70 -40 -10]
      | sbobj.Groups.Signals(2).Name = 'alpha'
      | sbobj.Groups.Signals(2).XData = [0 5 7.2 7.8 10 12.5 14 20]
      | sbobj.Groups.Signals(2).YData = [7 10 40 40 20 10.68 10 10]
      | sbobj.Groups.Signals(3).Name = 'beta'
      | sbobj.Groups.Signals(3).XData = [0 20]
      | sbobj.Groups.Signals(3).YData = [0 0]
      | sbobj.Groups.Signals(4).Name = 'speed brake'
      | sbobj.Groups.Signals(4).XData = [0 20]
      | sbobj.Groups.Signals(4).YData = [0 0]
      | sbobj.Groups.Signals(5).Name = 'LandingGear_down'
      | sbobj.Groups.Signals(5).XData = [0 20]
      | sbobj.Groups.Signals(5).YData = [1 1]
      | sbobj.Groups.TimeRange = [0 20]
  mu : Outport  Tag=STV Outport  VectorParamsAs1DForOutWhenUnconnected=off
  alpha : Outport  Tag=STV Outport  Port=2  VectorParamsAs1DForOutWhenUnconnected=off
  beta : Outport  Tag=STV Outport  Port=3  VectorParamsAs1DForOutWhenUnconnected=off
  speed brake : Outport  Tag=STV Outport  Port=4
  LandingGear_down : Outport  Tag=STV Outport  Port=5
  wires:
  Demux/5 -> LandingGear_down/1
  Demux/4 -> speed brake/1
  Demux/3 -> beta/1
  Demux/2 -> alpha/1
  Demux/1 -> mu/1
  FromWs/1 -> Demux/1

== system NDI/F-16 Vehicle Systems Model/Pilot commands storehouse/trun(deg) 初始高度10000ft 初始速度650ft//s攻角40度1 ==
  Demux : Demux  Tag=STV Demux  Outputs=5
      settings: DisplayOption=none
  FromWs : FromWorkspace  Tag=STV FromWs  VariableName=tuvar
      SigBuilderData=|
      | common.afterFinalStr = 'Extrapolate'
      | common.sampleTime = 0
      | dataSet.timeRange = [0 20]
      | dataSet.name = 'Group 5'
      | sbobj.Groups.Name = 'Group 5'
      | sbobj.Groups.Signals(1).Name = 'mu'
      | sbobj.Groups.Signals(1).XData = [0 2 5.5 6 7.2 8.5 10 12 15 20]
      | sbobj.Groups.Signals(1).YData = [0 0 -10 -140 -160 -160 -150 -70 -40 -10]
      | sbobj.Groups.Signals(2).Name = 'alpha'
      | sbobj.Groups.Signals(2).XData = [0 5 7.2 7.8 10 12.5 14 20]
      | sbobj.Groups.Signals(2).YData = [7 10 40 40 20 10.68 10 10]
      | sbobj.Groups.Signals(3).Name = 'beta'
      | sbobj.Groups.Signals(3).XData = [0 20]
      | sbobj.Groups.Signals(3).YData = [0 0]
      | sbobj.Groups.Signals(4).Name = 'speed brake'
      | sbobj.Groups.Signals(4).XData = [0 20]
      | sbobj.Groups.Signals(4).YData = [0 0]
      | sbobj.Groups.Signals(5).Name = 'LandingGear_down'
      | sbobj.Groups.Signals(5).XData = [0 20]
      | sbobj.Groups.Signals(5).YData = [1 1]
      | sbobj.Groups.TimeRange = [0 20]
  mu : Outport  Tag=STV Outport  VectorParamsAs1DForOutWhenUnconnected=off
  alpha : Outport  Tag=STV Outport  Port=2  VectorParamsAs1DForOutWhenUnconnected=off
  beta : Outport  Tag=STV Outport  Port=3  VectorParamsAs1DForOutWhenUnconnected=off
  speed brake : Outport  Tag=STV Outport  Port=4
  LandingGear_down : Outport  Tag=STV Outport  Port=5
  wires:
  Demux/5 -> LandingGear_down/1
  Demux/4 -> speed brake/1
  Demux/3 -> beta/1
  Demux/2 -> alpha/1
  Demux/1 -> mu/1
  FromWs/1 -> Demux/1

== system NDI/F-16 Vehicle Systems Model/Pilot commands storehouse/trun(deg) 初始高度10000ft 初始速度750ft//s攻角40度 ==
  Demux : Demux  Tag=STV Demux  Outputs=5
      settings: DisplayOption=none
  FromWs : FromWorkspace  Tag=STV FromWs  VariableName=tuvar
      SigBuilderData=|
      | common.afterFinalStr = 'Extrapolate'
      | common.sampleTime = 0
      | dataSet.timeRange = [0 20]
      | dataSet.name = 'Group 5'
      | sbobj.Groups.Name = 'Group 5'
      | sbobj.Groups.Signals(1).Name = 'mu'
      | sbobj.Groups.Signals(1).XData = [0 2 5.5 6 7.2 8.5 10 12 15 20]
      | sbobj.Groups.Signals(1).YData = [0 0 0 -150 -170 -170 -160 -70 -40 -10]
      | sbobj.Groups.Signals(2).Name = 'alpha'
      | sbobj.Groups.Signals(2).XData = [0 5 7.2 7.8 10 12.5 14 20]
      | sbobj.Groups.Signals(2).YData = [7 10 40 40 20 10.68 10 10]
      | sbobj.Groups.Signals(3).Name = 'beta'
      | sbobj.Groups.Signals(3).XData = [0 20]
      | sbobj.Groups.Signals(3).YData = [0 0]
      | sbobj.Groups.Signals(4).Name = 'speed brake'
      | sbobj.Groups.Signals(4).XData = [0 20]
      | sbobj.Groups.Signals(4).YData = [0 0]
      | sbobj.Groups.Signals(5).Name = 'LandingGear_down'
      | sbobj.Groups.Signals(5).XData = [0 20]
      | sbobj.Groups.Signals(5).YData = [1 1]
      | sbobj.Groups.TimeRange = [0 20]
  mu : Outport  Tag=STV Outport  VectorParamsAs1DForOutWhenUnconnected=off
  alpha : Outport  Tag=STV Outport  Port=2  VectorParamsAs1DForOutWhenUnconnected=off
  beta : Outport  Tag=STV Outport  Port=3  VectorParamsAs1DForOutWhenUnconnected=off
  speed brake : Outport  Tag=STV Outport  Port=4
  LandingGear_down : Outport  Tag=STV Outport  Port=5
  wires:
  Demux/5 -> LandingGear_down/1
  Demux/4 -> speed brake/1
  Demux/3 -> beta/1
  Demux/2 -> alpha/1
  Demux/1 -> mu/1
  FromWs/1 -> Demux/1
